simulink model "mcb_microchip_pmsm_parameter_est_SAME70"  (R2023b)
settings: Solver=FixedStepDiscrete  StartTime=0.0  StopTime=15  RelTol=1e-3  EnableMultiTasking=on
InitFcn:
  | mcb_microchip_pmsm_parameter_est_SAME70_data;
values from neighbouring files (symbols this model uses):
  Ts = T_pwm    (= 5e-05)    [mcb_microchip_pmsm_parameter_est_SAME70_data.m]
  Ts_motor = T_pwm/2    (= 2.5e-05)    [mcb_microchip_pmsm_parameter_est_SAME70_data.m]
undefined symbols (not defined in the file or in its folder): A24, AD10, AD7, ADC0, inverter, LQFP144, MaxPer, ms, ns, PA0, PA1, PA10, PA11, PA12, PA13, PA16, PA18, PA9, PB0, PD18, PD19, PD24, PD25, PD26, PI_params, Pin, pmsm, Resol, SAME70Q21B, target, Unsigned
libraries: simulink x18, MCHP_Blockset x13, mcbpmsmparamestlib x5, svdutilitieslib x4, mcbpositiondecoderlib x3, mcbplantlib x1, autolibpmsmexterior x1, mcbcontrolslib x1
(part 2 of 4)

== system mcb_microchip_pmsm_parameter_est_SAME70/Microcontroller/Configurations ==
  note: PIM: https://www.microchip.com/Developmenttools/ProductDetails/MA320203
  note: MCLV-2				SAME70-PIM
      | --------------------------------------------------
      | DBG_LED1			PC23
      | DBG_LED2			PA24
      |
      | Rx					PA09_URXD0
      | Tx					PA10_UTXD0
      |
      | HALLA				PA00 - PD13
      | HALLB				PA01 - PD10
      | HALLC				PA16 - PD11
      |
      | PWM1				PD24 (L) - PA11 (H)
      | PWM2				PD25 (L) - PA12 (H)
      | PWM3				PD26 (L) - PA13 (H)
      |
      | FAULT				PD09_FAULT_PWM
      |
      | POT				PB00 (not ok on early PIMs)
      | PUSH S2			PC03
      | PUSH S3			PC01
      |
      | PIM_V_M1			PD30
      | PIM_V_M2			PA17
      | PIM_V_M3			PA21 - PA19
  Compiler Options : MCHP_Blockset/System Configuration/Compiler Options  Priority=1  LATEST_CMPLR=on  COMP_LIST=Dynamic Options  COMP_LIST_TXT=xc32 - v4.30  DFP_LIST=Dynamic Options  DFP_LIST_TXT=from compiler  CMSIS_DSP=Dynamic Options  CMSIS_DSP_TXT=Not used  USE_64BIT_DOUBLE=off  MCHP_MULTITHREAD_COMPILATION=on  UseCustom_LinkerScript=off  MCHP_MASTERLINK=mcb_microchip_pmsm_parameter_est_SAME70_23b_lib/Microcontroller/Configurations/Microchip Master  OPTIMIZATION_LEVEL=2  MPLAB_LINKLIB=default  MPLAB_LINKLIB1=default  CodeReplacement=Dynamic Options  CodeReplacement_TXT=None  OPTIMIZATION_FLTO=off  OPTIMIZATION_REORDER=off  UNROLL_LOOPS=off  PROCEDURAL_ABSTRACTION=off  MCODE=is less than 32768 (faster)  MCONST=in data memory  MDATA=Use only memory below address 8192 (faster)  MSCALAR=Use only memory below address 8192 (faster)  MLARGEARRAY=off  MAGGREGATE=off  HEAP_SIZE=0  OMF=elf  DEBUG_INFO=on  ProduceHexOutput=off  AssemblyListing=off  SaveTemps=off  NO_EDS_WARN=on  PRINT_STATISTICS=off
      settings: SourceProductName=MPLAB Device Blocks for Simulink
  Microchip Master : MCHP_Blockset/System Configuration/Microchip Master  Priority=1  PICREF=SAME70Q21B - LQFP144  TIMESTEP_REF="ADC0  ( 0.001s )"  BUSYFLAG=Dynamic Options  BUSYFLAG_TXT=A24 / Pin[56]  VDD_range=Dynamic Options  PWRTEN=Not used  BOREN=Disable  BODENV=2.7V  BORV=Not used  FPWRT=64ms  DSBOREN=Enable ZPBOR during Deep Sleep Mode  DSLPBOR=Not used  MCLRE=Enabled  SMCLR=MCLR pin generates a normal system Reset  PMDL1WAY=Allow only one reconfiguration  RSTPRI=Device will obtain reset instruction from Primary flash  TEMP=Not used  SOSCSRC=Not used  SOSCSEL=Not used  IOL1WAY=Allow only one reconfiguration  ALTVREF=Not used  DISUVREG=Not used  DSSWEN=Not used  LPCFG=Not used  RTCBAT=Not used  VBTBOR=Not used  WUTSEL=Not used  POWERSAVE=off  FNOSC=Fast RC Osc w/Div-by-N (FRCDIV)  FPR=ECIO w/ PLL 16x  FOSFPR=HS3 w/PLL 16x  FOS=Internal Fast RC  FRANGE=High Range  OSCILLATOR_SELECT=Crystal / Ceramic resonator  OSCILLATOR_SELECT_spd=Crystal / Ceramic resonator  QUARTZ=12e6  QUARTZ_spd=12e6  POSCGAIN=2x gain setting  POSCBOOST=Boost the kick start of the oscillator  SOSCGAIN=2x gain setting  SOSCBOOST=Boost the kick start of the oscillator  ACTIV_PLL=on  ACTIV_PLL_spd=on  MIPS_DESIRED=300e6  MIPS_DESIRED_spd=300e6  CPUDIV=Divide by 1  FPLLMUL=Not used  FPLLIDIV=8x Divider  POSCFREQ=Not used  POSCMD=Primary Oscillator Disabled  POSCMOD=Primary osc disabled  MIPS=300 * 1e6  ACLKCON=Optimized for PWM resolution & ADC conversion speed  ACLKCON_spd=Optimized for PWM resolution & ADC conversion speed  FPLLODIV=32x Divider  PLLKEN=Clock switch to PLL source will wait until the PLL lock signal is valid  FCKSM=Clock Switch Disabled; FSCM Disabled  FCKSMEN=Sw Disabled; Mon Disabled  IESO=Enabled  DSWDTPS=1:2^36  FWDTEN=Disable  FWDTWINSZ=Window size is 25%  FWPSA=1:512  FWPSA0=1:128  FWPSB=1:16  WDT=Disable  WDTPOST=1:32768  WDTPRE=1:128  WDTPS=1:1048576  WINDIS=Watchdog Timer is in non-Window mode  WWDTEN=Non-Window mode  DSWDTEN=Enable DSWDT during Deep Sleep Mode  DSWDTOSC=Select LPRC as DSWDT Reference clock  FWDT_RCLKSEL=WDT Run Mode uses BFRC:256  FWDT_RWDTPS=1:2147483648  FWDT_SWDTMPS=1:2147483648  FWDT_WDTEN=WDT is controlled by software; use WDTCON.ON bit  FWDT_WDTRSTEN=WDT event generates a reset  FWDT_WDTWIN=WDT Window is 25% of WDT period  FWDT_WINEN=Watchdog Timer operates in Window mode  FPBDIV=Not used  FSOSCEN=Disable Secondary Oscillator  LPRCSEL=Not used  OSCIOFCN=Not used  OSCIOFNC=OSC2 is clock output  LVRCFG=Not used  PLL_96MHZ=Not used  PLL96MHZ=Not used  PLLDIV=Not used  WDTCLK=Not used  WDTCMX=Not used  WDTWIN=WDT Window is 25% of WDT period  XTCFG=24-32 MHz crystals  XTBST=Boost the kick-start  APL=Aux Flash Code protect is disabled  APLK=Aux Flash Write Protection or Code Protection is Enabled  AWRP=Auxiliary program memory is not write-protected  BSS=No Boot program Flash segment  BWP=Not used  BWRP=Boot Segment may be written  CP=Protection Disabled  EBS=No Boot EEPROM  ESS=No Segment Data EEPROM  GCP=Disable  GSS=High Security Code Protection Enabled  GSS0=Not used  GSSK=General Segment Write Protection or Code Protection is Enabled  GWRP=Disable  PWP=Not used  RBS=No Boot RAM  RSS=No Secure RAM  SSS=No Secure Segment  SWRP=Secure segment may be written  WPCFG=Not used  WPDIS=Not used  WPEND=Not used  WPFP=Not used  ICESEL=Communicate on PGEC1/PGED1  ICS=Use PGC/EMUC and PGD/EMUD  JTAGEN=Disable  FICD_JTAGEN=Disable  COE=Not used  RES=Not used  DEBUG=Debugger is disabled  BACKBUG=Not used  BKBUG=Not used  ALTI2C=I2C mapped to SDA1/SCL1 pins  ALTI2C1=I2C1 mapped to SDA1/SCL1 pins  ALTI2C2=I2C2 mapped to SDA2/SCL2 pins  ALTI2C3=I2C3 mapped to SDA3/SCL3 pins  FDEVOPT1_ALTI2C1=Primary I2C1 pins are used  FDEVOPT1_ALTI2C2=Primary I2C2 pins are used  FDEVOPT1_SPI2MAPDIS=SPI2 pins are selected by peripheral pin selection feature  ALTQIO=QEA1; QEB1; INDX1 are selected as inputs to QEI1  ALTSS1=SS1A is selected as the I/O pin for SPI1  CMPPOL0=Hysteresis is applied to falling edge  CMPPOL1=Hysteresis is applied to falling edge  FCANIO=Not used  FETHIO=Default Ethernet I/O  FMIIEN=MII Enabled  FSRSSEL=Not used  FUSBIDIO=Controlled by the USB Module  FVBUSONIO=Not used  HPOL=Active High  HYST0=45 mV Hysteresis  HYST1=45 mV Hysteresis  I2C1SEL=Not used  LPOL=Active High  PWMPIN=Control with PORT/TRIS regs  RTCOSC=Not used  UPLLEN=USB PLL Disabled  UPLLIDIV=Not used  ATMOD8=Not used  ALTPMP=Not used  I2C2SEL=Not used  ALTADREF=Not used  ALTCVREF=Not used  PWMLOCK=PWM registers may be written without key sequence  INT_PRIORITY_DMA=7  MCHP_TIMER_RESULT=[1 98.999999999999971578 ]  MCHP_PORT={Busy Flag}{Busy}0:1:A24;  MCHP_PLLRegisters=[-1 -1 -1 -1 -1]  MCHPVAR=MCHP.id.name='SAME70Q21B';MCHP.id.N=reshape([70 21 -1],1,3);MCHP.id.L=reshape({ 'SAME','Q','B'},1,3);MCHP.id.maskset='';MCHP.id.dos='';MCHP.id.ds='';MCHP.id.archTxt='';MCHP.id.clonedfrom='';MCHP.id.Arch=5;MCHP.id.pinout=reshape({ 'LFBGA144','UFBGA144','LQFP144'},1,3);MCHP.Rx=reshape([102 21 11 1 4 99 20 38 132 6 93 26 39 131 7 91 31 40 128 10 77 105 41 126 27 73 109 58 125 28 114 79 54 121 -1 35 89 48 119 -1 36 141 82 113 -1 75 142 86 110 -1 66 -1 90 101 -1 64 -1 94 98 -1 68 87 17 92 -1 42 144 19 88 -1 51 -1 97 84 -1 49 -1 18 106 -1 45 -1 100 78 -1 25 -1 103 74 -1 24 -1 111 69 -1 23 -1 117 67 -1 22 -1 120 65 -1 32 -1 122 63 -1 37 -1 124 60 -1 46 -1 127 57 -1 56 -1 130 55 -1 59 -1 133 52 -1 62 -1 13 53 -1 70 -1 12 47 -1 112 -1 76 71 -1 129 -1 16 108 -1 116 -1 15 34 -1 118 -1 14 2 -1],5,32);MCHP.memory.PERIPHERALS.size=MCHP_Fun.Hex2num('41C0000000000000');MCHP.memory.SYSTEM.size=MCHP_Fun.Hex2num('41B0000000000000');MCHP.memory.QSPIMEM.size=MCHP_Fun.Hex2num('41C0000000000000');MCHP.memory.AXIMX.size=1048576;MCHP.memory.ITCM.size=2097152;MCHP.memory.IFLASH.size=2097152;MCHP.memory.IROM.size=16384;MCHP.memory.DTCM.size=131072;MCHP.memory.IRAM.size=393216;MCHP.memory.EBI_CS0.size=16777216;MCHP.memory.EBI_CS1.size=16777216;MCHP.memory.EBI_CS2.size=16777216;MCHP.memory.EBI_CS3.size=16777216;MCHP.module.SUPC.PID=0;MCHP.module.SUPC.vector='SUPC';MCHP.module.SUPC.pin.WKUP0.txt={ 'PA0'};MCHP.module.SUPC.pin.WKUP0.Rx_idx=0;MCHP.module.SUPC.pin.WKUP0.ABCD=-2;MCHP.module.SUPC.pin.WKUP1.txt={ 'PA1'};MCHP.module.SUPC.pin.WKUP1.Rx_idx=1;MCHP.module.SUPC.pin.WKUP1.ABCD=-2;MCHP.module.SUPC.pin.WKUP2.txt={ 'PA2'};MCHP.module.SUPC.pin.WKUP2.Rx_idx=2;MCHP.module.SUPC.pin.WKUP2.ABCD=-2;MCHP.module.SUPC.pin.WKUP3.txt={ 'PA4'};MCHP.module.SUPC.pin.WKUP3.Rx_idx=4;MCHP.module.SUPC.pin.WKUP3.ABCD=-2;MCHP.module.SUPC.pin.WKUP4.txt={ 'PA5'};MCHP.module.SUPC.pin.WKUP4.Rx_idx=5;MCHP.module.SUPC.pin.WKUP4.ABCD=-2;MCHP.module.SUPC.pin.WKUP6.txt={ 'PA9'};MCHP.module.SUPC.pin.WKUP6.Rx_idx=9;MCHP.module.SUPC.pin.WKUP6.ABCD=-2;MCHP.module.SUPC.pin.WKUP7.txt={ 'PA11'};MCHP.module.SUPC.pin.WKUP7.Rx_idx=11;MCHP.module.SUPC.pin.WKUP7.ABCD=-2;MCHP.module.SUPC.pin.WKUP8.txt={ 'PA14'};MCHP.module.SUPC.pin.WKUP8.Rx_idx=14;MCHP.module.SUPC.pin.WKUP8.ABCD=-2;MCHP.module.SUPC.pin.WKUP9.txt={ 'PA19'};MCHP.module.SUPC.pin.WKUP9.Rx_idx=19;MCHP.module.SUPC.pin.WKUP9.ABCD=-2;MCHP.module.SUPC.pin.WKUP10.txt={ 'PA20'};MCHP.module.SUPC.pin.WKUP10.Rx_idx=20;MCHP.module.SUPC.pin.WKUP10.ABCD=-2;MCHP.module.SUPC.pin.WKUP11.txt={ 'PA30'};MCHP.module.SUPC.pin.WKUP11.Rx_idx=30;MCHP.module.SUPC.pin.WKUP11.ABCD=-2;MCHP.module.SUPC.pin.WKUP12.txt={ 'PB3'};MCHP.module.SUPC.pin.WKUP12.Rx_idx=35;MCHP.module.SUPC.pin.WKUP12.ABCD=-2;MCHP.module.SUPC.pin.WKUP13.txt={ 'PB5'};MCHP.module.SUPC.pin.WKUP13.Rx_idx=37;MCHP.module.SUPC.pin.WKUP13.ABCD=-2;MCHP.module.SUPC.pin.WKUP5.txt={ 'PD28'};MCHP.module.SUPC.pin.WKUP5.Rx_idx=124;MCHP.module.SUPC.pin.WKUP5.ABCD=-2;MCHP.module.RSTC.PID=1;MCHP.module.RSTC.vector='RSTC';MCHP.module.RTC.PID=2;MCHP.module.RTC.vector='RTC';MCHP.module.RTC.pin.RTCOUT0.txt={ 'PB0'};MCHP.module.RTC.pin.RTCOUT0.Rx_idx=32;MCHP.module.RTC.pin.RTCOUT0.ABCD=-2;MCHP.module.RTC.pin.RTCOUT1.txt={ 'PB1'};MCHP.module.RTC.pin.RTCOUT1.Rx_idx=33;MCHP.module.RTC.pin.RTCOUT1.ABCD=-2;MCHP.module.RTT.PID=3;MCHP.module.RTT.vector='RTT';MCHP.module.WDT.PID=4;MCHP.module.WDT.vector='WDT';MCHP.module.PMC.PID=5;MCHP.module.PMC.vector='PMC';MCHP.module.PMC.pin.PCK0.txt=reshape({ 'PA6','PB12','PB13'},1,3);MCHP.module.PMC.pin.PCK0.Rx_idx=reshape([6 44 45],1,3);MCHP.module.PMC.pin.PCK0.ABCD=reshape([1 3 1],1,3);MCHP.module.PMC.pin.PCK1.txt=reshape({ 'PA17','PA21'},1,2);MCHP.module.PMC.pin.PCK1.Rx_idx=reshape([17 21],1,2);MCHP.module.PMC.pin.PCK1.ABCD=reshape([1 1],1,2);MCHP.module.PMC.pin.PCK2.txt=reshape({ 'PA3','PA18','PA31','PB3','PD31'},1,5);MCHP.module.PMC.pin.PCK2.Rx_idx=reshape([3 18 31 35 127],1,5);MCHP.module.PMC.pin.PCK2.ABCD=reshape([2 1 1 1 2],1,5);MCHP.module.PMC.pin.XIN.txt={ 'PB9'};MCHP.module.PMC.pin.XIN.Rx_idx=41;MCHP.module.PMC.pin.XIN.ABCD=-2;MCHP.module.PMC.pin.XOUT.txt={ 'PB8'};MCHP.module.PMC.pin.XOUT.Rx_idx=40;MCHP.module.PMC.pin.XOUT.ABCD=-2;MCHP.module.PMC.pin.XIN32.txt={ 'PA7'};MCHP.module.PMC.pin.XIN32.Rx_idx=7;MCHP.module.PMC.pin.XIN32.ABCD=-2;MCHP.module.PMC.pin.XOUT32.txt={ 'PA8'};MCHP.module.PMC.pin.XOUT32.Rx_idx=8;MCHP.module.PMC.pin.XOUT32.ABCD=-2;MCHP.module.EFC.PID=6;MCHP.module.EFC.vector='EFC';MCHP.module.EFC.pin.ERASE.txt={ 'PB12'};MCHP.module.EFC.pin.ERASE.Rx_idx=44;MCHP.module.EFC.pin.ERASE.ABCD=-2;MCHP.module.UART0.PID=7;MCHP.module.UART0.vector='UART0';MCHP.module.UART0.pin.URXD0.txt={ 'PA9'};MCHP.module.UART0.pin.URXD0.Rx_idx=9;MCHP.module.UART0.pin.URXD0.ABCD=0;MCHP.module.UART0.pin.UTXD0.txt={ 'PA10'};MCHP.module.UART0.pin.UTXD0.Rx_idx=10;MCHP.module.UART0.pin.UTXD0.ABCD=0;MCHP.module.UART1.PID=8;MCHP.module.UART1.vector='UART1';MCHP.module.UART1.pin.URXD1.txt={ 'PA5'};MCHP.module.UART1.pin.URXD1.Rx_idx=5;MCHP.module.UART1.pin.URXD1.ABCD=2;MCHP.module.UART1.pin.UTXD1.txt=reshape({ 'PA4','PA6','PD26'},1,3);MCHP.module.UART1.pin.UTXD1.Rx_idx=reshape([4 6 122],1,3);MCHP.module.UART1.pin.UTXD1.ABCD=reshape([2 2 3],1,3);MCHP.module.PIOA.PID=10;MCHP.module.PIOA.vector='PIOA';MCHP.module.PIOA.pin.PIODC0.txt={ 'PA3'};MCHP.module.PIOA.pin.PIODC0.Rx_idx=3;MCHP.module.PIOA.pin.PIODC0.ABCD=-2;MCHP.module.PIOA.pin.PIODC1.txt={ 'PA4'};MCHP.module.PIOA.pin.PIODC1.Rx_idx=4;MCHP.module.PIOA.pin.PIODC1.ABCD=-2;MCHP.module.PIOA.pin.PIODC2.txt={ 'PA5'};MCHP.module.PIOA.pin.PIODC2.Rx_idx=5;MCHP.module.PIOA.pin.PIODC2.ABCD=-2;MCHP.module.PIOA.pin.PIODC3.txt={ 'PA9'};MCHP.module.PIOA.pin.PIODC3.Rx_idx=9;MCHP.module.PIOA.pin.PIODC3.ABCD=-2;MCHP.module.PIOA.pin.PIODC4.txt={ 'PA10'};MCHP.module.PIOA.pin.PIODC4.Rx_idx=10;MCHP.module.PIOA.pin.PIODC4.ABCD=-2;MCHP.module.PIOA.pin.PIODC5.txt={ 'PA11'};MCHP.module.PIOA.pin.PIODC5.Rx_idx=11;MCHP.module.PIOA.pin.PIODC5.ABCD=-2;MCHP.module.PIOA.pin.PIODC6.txt={ 'PA12'};MCHP.module.PIOA.pin.PIODC6.Rx_idx=12;MCHP.module.PIOA.pin.PIODC6.ABCD=-2;MCHP.module.PIOA.pin.PIODC7.txt={ 'PA13'};MCHP.module.PIOA.pin.PIODC7.Rx_idx=13;MCHP.module.PIOA.pin.PIODC7.ABCD=-2;MCHP.module.PIOA.pin.PIODCEN1.txt={ 'PA14'};MCHP.module.PIOA.pin.PIODCEN1.Rx_idx=14;MCHP.module.PIOA.pin.PIODCEN1.ABCD=-2;MCHP.module.PIOA.pin.PIODCEN2.txt={ 'PA21'};MCHP.module.PIOA.pin.PIODCEN2.Rx_idx=21;MCHP.module.PIOA.pin.PIODCEN2.ABCD=-2;MCHP.module.PIOA.pin.PIODCCLK.txt={ 'PA22'};MCHP.module.PIOA.pin.PIODCCLK.Rx_idx=22;MCHP.module.PIOA.pin.PIODCCLK.ABCD=-2;MCHP.module.PIOB.PID=11;MCHP.module.PIOB.vector='PIOB';MCHP.module.PIOC.PID=12;MCHP.module.PIOC.vector='PIOC';MCHP.module.USART0.PID=13;MCHP.module.USART0.vector='USART0';MCHP.module.USART0.pin.CTS0.txt={ 'PB2'};MCHP.module.USART0.pin.CTS0.Rx_idx=34;MCHP.module.USART0.pin.CTS0.ABCD=2;MCHP.module.USART0.pin.DCD0.txt={ 'PD0'};MCHP.module.USART0.pin.DCD0.Rx_idx=96;MCHP.module.USART0.pin.DCD0.ABCD=3;MCHP.module.USART0.pin.DSR0.txt={ 'PD2'};MCHP.module.USART0.pin.DSR0.Rx_idx=98;MCHP.module.USART0.pin.DSR0.ABCD=3;MCHP.module.USART0.pin.DTR0.txt={ 'PD1'};MCHP.module.USART0.pin.DTR0.Rx_idx=97;MCHP.module.USART0.pin.DTR0.ABCD=3;MCHP.module.USART0.pin.RI0.txt={ 'PD3'};MCHP.module.USART0.pin.RI0.Rx_idx=99;MCHP.module.USART0.pin.RI0.ABCD=3;MCHP.module.USART0.pin.RTS0.txt={ 'PB3'};MCHP.module.USART0.pin.RTS0.Rx_idx=35;MCHP.module.USART0.pin.RTS0.ABCD=2;MCHP.module.USART0.pin.RXD0.txt={ 'PB0'};MCHP.module.USART0.pin.RXD0.Rx_idx=32;MCHP.module.USART0.pin.RXD0.ABCD=2;MCHP.module.USART0.pin.SCK0.txt={ 'PB13'};MCHP.module.USART0.pin.SCK0.Rx_idx=45;MCHP.module.USART0.pin.SCK0.ABCD=2;MCHP.module.USART0.pin.TXD0.txt={ 'PB1'};MCHP.module.USART0.pin.TXD0.Rx_idx=33;MCHP.module.USART0.pin.TXD0.ABCD=2;MCHP.module.USART1.PID=14;MCHP.module.USART1.vector='USART1';MCHP.module.USART1.pin.CTS1.txt={ 'PA25'};MCHP.module.USART1.pin.CTS1.Rx_idx=25;MCHP.module.USART1.pin.CTS1.ABCD=0;MCHP.module.USART1.pin.DCD1.txt={ 'PA26'};MCHP.module.USART1.pin.DCD1.Rx_idx=26;MCHP.module.USART1.pin.DCD1.ABCD=0;MCHP.module.USART1.pin.DSR1.txt={ 'PA28'};MCHP.module.USART1.pin.DSR1.Rx_idx=28;MCHP.module.USART1.pin.DSR1.ABCD=0;MCHP.module.USART1.pin.DTR1.txt={ 'PA27'};MCHP.module.USART1.pin.DTR1.Rx_idx=27;MCHP.module.USART1.pin.DTR1.ABCD=0;MCHP.module.USART1.pin.LONCOL1.txt={ 'PA3'};MCHP.module.USART1.pin.LONCOL1.Rx_idx=3;MCHP.module.USART1.pin.LONCOL1.ABCD=1;MCHP.module.USART1.pin.RI1.txt={ 'PA29'};MCHP.module.USART1.pin.RI1.Rx_idx=29;MCHP.module.USART1.pin.RI1.ABCD=0;MCHP.module.USART1.pin.RTS1.txt={ 'PA24'};MCHP.module.USART1.pin.RTS1.Rx_idx=24;MCHP.module.USART1.pin.RTS1.ABCD=0;MCHP.module.USART1.pin.RXD1.txt={ 'PA21'};MCHP.module.USART1.pin.RXD1.Rx_idx=21;MCHP.module.USART1.pin.RXD1.ABCD=0;MCHP.module.USART1.pin.SCK1.txt={ 'PA23'};MCHP.module.USART1.pin.SCK1.Rx_idx=23;MCHP.module.USART1.pin.SCK1.ABCD=0;MCHP.module.USART1.pin.TXD1.txt={ 'PB4'};MCHP.module.USART1.pin.TXD1.Rx_idx=36;MCHP.module.USART1.pin.TXD1.ABCD=3;MCHP.module.USART2.PID=15;MCHP.module.USART2.vector='USART2';MCHP.module.USART2.pin.CTS2.txt={ 'PD19'};MCHP.module.USART2.pin.CTS2.Rx_idx=115;MCHP.module.USART2.pin.CTS2.ABCD=1;MCHP.module.USART2.pin.DCD2.txt={ 'PD4'};MCHP.module.USART2.pin.DCD2.Rx_idx=100;MCHP.module.USART2.pin.DCD2.ABCD=3;MCHP.module.USART2.pin.DSR2.txt={ 'PD6'};MCHP.module.USART2.pin.DSR2.Rx_idx=102;MCHP.module.USART2.pin.DSR2.ABCD=3;MCHP.module.USART2.pin.DTR2.txt={ 'PD5'};MCHP.module.USART2.pin.DTR2.Rx_idx=101;MCHP.module.USART2.pin.DTR2.ABCD=3;MCHP.module.USART2.pin.RI2.txt={ 'PD7'};MCHP.module.USART2.pin.RI2.Rx_idx=103;MCHP.module.USART2.pin.RI2.ABCD=3;MCHP.module.USART2.pin.RTS2.txt={ 'PD18'};MCHP.module.USART2.pin.RTS2.Rx_idx=114;MCHP.module.USART2.pin.RTS2.ABCD=1;MCHP.module.USART2.pin.RXD2.txt={ 'PD15'};MCHP.module.USART2.pin.RXD2.Rx_idx=111;MCHP.module.USART2.pin.RXD2.ABCD=1;MCHP.module.USART2.pin.SCK2.txt={ 'PD17'};MCHP.module.USART2.pin.SCK2.Rx_idx=113;MCHP.module.USART2.pin.SCK2.ABCD=1;MCHP.module.USART2.pin.TXD2.txt={ 'PD16'};MCHP.module.USART2.pin.TXD2.Rx_idx=112;MCHP.module.USART2.pin.TXD2.ABCD=1;MCHP.module.PIOD.PID=16;MCHP.module.PIOD.vector='PIOD';MCHP.module.PIOE.PID=17;MCHP.module.PIOE.vector='PIOE';MCHP.module.HSMCI.PID=18;MCHP.module.HSMCI.vector='HSMCI';MCHP.module.HSMCI.pin.MCCDA.txt={ 'PA28'};MCHP.module.HSMCI.pin.MCCDA.Rx_idx=28;MCHP.module.HSMCI.pin.MCCDA.ABCD=2;MCHP.module.HSMCI.pin.MCCK.txt={ 'PA25'};MCHP.module.HSMCI.pin.MCCK.Rx_idx=25;MCHP.module.HSMCI.pin.MCCK.ABCD=3;MCHP.module.HSMCI.pin.MCDA0.txt={ 'PA30'};MCHP.module.HSMCI.pin.MCDA0.Rx_idx=30;MCHP.module.HSMCI.pin.MCDA0.ABCD=2;MCHP.module.HSMCI.pin.MCDA1.txt={ 'PA31'};MCHP.module.HSMCI.pin.MCDA1.Rx_idx=31;MCHP.module.HSMCI.pin.MCDA1.ABCD=2;MCHP.module.HSMCI.pin.MCDA2.txt={ 'PA26'};MCHP.module.HSMCI.pin.MCDA2.Rx_idx=26;MCHP.module.HSMCI.pin.MCDA2.ABCD=2;MCHP.module.HSMCI.pin.MCDA3.txt={ 'PA27'};MCHP.module.HSMCI.pin.MCDA3.Rx_idx=27;MCHP.module.HSMCI.pin.MCDA3.ABCD=2;MCHP.module.TWIHS0.PID=19;MCHP.module.TWIHS0.vector='TWIHS0';MCHP.module.TWIHS0.pin.TWCK0.txt={ 'PA4'};MCHP.module.TWIHS0.pin.TWCK0.Rx_idx=4;MCHP.module.TWIHS0.pin.TWCK0.ABCD=0;MCHP.module.TWIHS0.pin.TWD0.txt={ 'PA3'};MCHP.module.TWIHS0.pin.TWD0.Rx_idx=3;MCHP.module.TWIHS0.pin.TWD0.ABCD=0;MCHP.module.TWIHS1.PID=20;MCHP.module.TWIHS1.vector='TWIHS1';MCHP.module.TWIHS1.pin.TWCK1.txt={ 'PB5'};MCHP.module.TWIHS1.pin.TWCK1.Rx_idx=37;MCHP.module.TWIHS1.pin.TWCK1.ABCD=0;MCHP.module.TWIHS1.pin.TWD1.txt={ 'PB4'};MCHP.module.TWIHS1.pin.TWD1.Rx_idx=36;MCHP.module.TWIHS1.pin.TWD1.ABCD=0;MCHP.module.SPI0.PID=21;MCHP.module.SPI0.vector='SPI0';MCHP.module.SPI0.pin.MISO.txt={ 'PD20'};MCHP.module.SPI0.pin.MISO.Rx_idx=116;MCHP.module.SPI0.pin.MISO.ABCD=1;MCHP.module.SPI0.pin.MOSI.txt={ 'PD21'};MCHP.module.SPI0.pin.MOSI.Rx_idx=117;MCHP.module.SPI0.pin.MOSI.ABCD=1;MCHP.module.SPI0.pin.NPCS0.txt={ 'PB2'};MCHP.module.SPI0.pin.NPCS0.Rx_idx=34;MCHP.module.SPI0.pin.NPCS0.ABCD=3;MCHP.module.SPI0.pin.NPCS1.txt=reshape({ 'PA31','PD25'},1,2);MCHP.module.SPI0.pin.NPCS1.Rx_idx=reshape([31 121],1,2);MCHP.module.SPI0.pin.NPCS1.ABCD=reshape([0 1],1,2);MCHP.module.SPI0.pin.NPCS2.txt={ 'PD12'};MCHP.module.SPI0.pin.NPCS2.Rx_idx=108;MCHP.module.SPI0.pin.NPCS2.ABCD=2;MCHP.module.SPI0.pin.NPCS3.txt={ 'PD27'};MCHP.module.SPI0.pin.NPCS3.Rx_idx=123;MCHP.module.SPI0.pin.NPCS3.ABCD=1;MCHP.module.SPI0.pin.SPCK.txt={ 'PD22'};MCHP.module.SPI0.pin.SPCK.Rx_idx=118;MCHP.module.SPI0.pin.SPCK.ABCD=1;MCHP.module.SSC.PID=22;MCHP.module.SSC.vector='SSC';MCHP.module.SSC.pin.RD.txt={ 'PA10'};MCHP.module.SSC.pin.RD.Rx_idx=10;MCHP.module.SSC.pin.RD.ABCD=2;MCHP.module.SSC.pin.RF.txt={ 'PD24'};MCHP.module.SSC.pin.RF.Rx_idx=120;MCHP.module.SSC.pin.RF.ABCD=1;MCHP.module.SSC.pin.RK.txt={ 'PA22'};MCHP.module.SSC.pin.RK.Rx_idx=22;MCHP.module.SSC.pin.RK.ABCD=0;MCHP.module.SSC.pin.TD.txt=reshape({ 'PB5','PD10','PD26'},1,3);MCHP.module.SSC.pin.TD.Rx_idx=reshape([37 106 122],1,3);MCHP.module.SSC.pin.TD.ABCD=reshape([3 2 1],1,3);MCHP.module.SSC.pin.TF.txt={ 'PB0'};MCHP.module.SSC.pin.TF.Rx_idx=32;MCHP.module.SSC.pin.TF.ABCD=3;MCHP.module.SSC.pin.TK.txt={ 'PB1'};MCHP.module.SSC.pin.TK.Rx_idx=33;MCHP.module.SSC.pin.TK.ABCD=3;MCHP.module.TC0(1).PID=23;MCHP.module.TC0(1).vector='TC0';MCHP.module.TC0(1).pin.TCLK0.txt={ 'PA4'};MCHP.module.TC0(1).pin.TCLK0.Rx_idx=4;MCHP.module.TC0(1).pin.TCLK0.ABCD=1;MCHP.module.TC0(1).pin.TCLK1.txt={ 'PA28'};MCHP.module.TC0(1).pin.TCLK1.Rx_idx=28;MCHP.module.TC0(1).pin.TCLK1.ABCD=1;MCHP.module.TC0(1).pin.TCLK2.txt={ 'PA29'};MCHP.module.TC0(1).pin.TCLK2.Rx_idx=29;MCHP.module.TC0(1).pin.TCLK2.ABCD=1;MCHP.module.TC0(1).pin.TIOA0.txt={ 'PA0'};MCHP.module.TC0(1).pin.TIOA0.Rx_idx=0;MCHP.module.TC0(1).pin.TIOA0.ABCD=1;MCHP.module.TC0(1).pin.TIOA1.txt={ 'PA15'};MCHP.module.TC0(1).pin.TIOA1.Rx_idx=15;MCHP.module.TC0(1).pin.TIOA1.ABCD=1;MCHP.module.TC0(1).pin.TIOA2.txt={ 'PA26'};MCHP.module.TC0(1).pin.TIOA2.Rx_idx=26;MCHP.module.TC0(1).pin.TIOA2.ABCD=1;MCHP.module.TC0(1).pin.TIOB0.txt={ 'PA1'};MCHP.module.TC0(1).pin.TIOB0.Rx_idx=1;MCHP.module.TC0(1).pin.TIOB0.ABCD=1;MCHP.module.TC0(1).pin.TIOB1.txt={ 'PA16'};MCHP.module.TC0(1).pin.TIOB1.Rx_idx=16;MCHP.module.TC0(1).pin.TIOB1.ABCD=1;MCHP.module.TC0(1).pin.TIOB2.txt={ 'PA27'};MCHP.module.TC0(1).pin.TIOB2.Rx_idx=27;MCHP.module.TC0(1).pin.TIOB2.ABCD=1;MCHP.module.TC0(2).PID=24;MCHP.module.TC0(2).vector='TC1';MCHP.module.TC0(2).pin=reshape(MCHP_Fun.Hex2num('[]'),0,0);MCHP.module.TC0(3).PID=25;MCHP.module.TC0(3).vector='TC2';MCHP.module.TC0(3).pin=reshape(MCHP_Fun.Hex2num('[]'),0,0);MCHP.module.TC1(1).PID=26;MCHP.module.TC1(1).vector='TC3';MCHP.module.TC1(1).pin.TCLK3.txt={ 'PC25'};MCHP.module.TC1(1).pin.TCLK3.Rx_idx=89;MCHP.module.TC1(1).pin.TCLK3.ABCD=1;MCHP.module.TC1(1).pin.TCLK4.txt={ 'PC28'};MCHP.module.TC1(1).pin.TCLK4.Rx_idx=92;MCHP.module.TC1(1).pin.TCLK4.ABCD=1;MCHP.module.TC1(1).pin.TCLK5.txt={ 'PC31'};MCHP.module.TC1(1).pin.TCLK5.Rx_idx=95;MCHP.module.TC1(1).pin.TCLK5.ABCD=1;MCHP.module.TC1(1).pin.TIOA3.txt={ 'PC23'};MCHP.module.TC1(1).pin.TIOA3.Rx_idx=87;MCHP.module.TC1(1).pin.TIOA3.ABCD=1;MCHP.module.TC1(1).pin.TIOA4.txt={ 'PC26'};MCHP.module.TC1(1).pin.TIOA4.Rx_idx=90;MCHP.module.TC1(1).pin.TIOA4.ABCD=1;MCHP.module.TC1(1).pin.TIOA5.txt={ 'PC29'};MCHP.module.TC1(1).pin.TIOA5.Rx_idx=93;MCHP.module.TC1(1).pin.TIOA5.ABCD=1;MCHP.module.TC1(1).pin.TIOB3.txt={ 'PC24'};MCHP.module.TC1(1).pin.TIOB3.Rx_idx=88;MCHP.module.TC1(1).pin.TIOB3.ABCD=1;MCHP.module.TC1(1).pin.TIOB4.txt={ 'PC27'};MCHP.module.TC1(1).pin.TIOB4.Rx_idx=91;MCHP.module.TC1(1).pin.TIOB4.ABCD=1;MCHP.module.TC1(1).pin.TIOB5.txt={ 'PC30'};MCHP.module.TC1(1).pin.TIOB5.Rx_idx=94;MCHP.module.TC1(1).pin.TIOB5.ABCD=1;MCHP.module.TC1(2).PID=27;MCHP.module.TC1(2).vector='TC4';MCHP.module.TC1(2).pin=reshape(MCHP_Fun.Hex2num('[]'),0,0);MCHP.module.TC1(3).PID=28;MCHP.module.TC1(3).vector='TC5';MCHP.module.TC1(3).pin=reshape(MCHP_Fun.Hex2num('[]'),0,0);MCHP.module.AFEC0.PID=29;MCHP.module.AFEC0.vector='AFEC0';MCHP.module.AFEC0.pin.ADTRG.txt={ 'PA8'};MCHP.module.AFEC0.pin.ADTRG.Rx_idx=8;MCHP.module.AFEC0.pin.ADTRG.ABCD=1;MCHP.module.AFEC0.pin.AD0.txt={ 'PD30'};MCHP.module.AFEC0.pin.AD0.Rx_idx=126;MCHP.module.AFEC0.pin.AD0.ABCD=-2;MCHP.module.AFEC0.pin.AD1.txt={ 'PA21'};MCHP.module.AFEC0.pin.AD1.Rx_idx=21;MCHP.module.AFEC0.pin.AD1.ABCD=-2;MCHP.module.AFEC0.pin.AD2.txt={ 'PB3'};MCHP.module.AFEC0.pin.AD2.Rx_idx=35;MCHP.module.AFEC0.pin.AD2.ABCD=-2;MCHP.module.AFEC0.pin.AD3.txt={ 'PE5'};MCHP.module.AFEC0.pin.AD3.Rx_idx=133;MCHP.module.AFEC0.pin.AD3.ABCD=-2;MCHP.module.AFEC0.pin.AD4.txt={ 'PE4'};MCHP.module.AFEC0.pin.AD4.Rx_idx=132;MCHP.module.AFEC0.pin.AD4.ABCD=-2;MCHP.module.AFEC0.pin.AD5.txt={ 'PB2'};MCHP.module.AFEC0.pin.AD5.Rx_idx=34;MCHP.module.AFEC0.pin.AD5.ABCD=-2;MCHP.module.AFEC0.pin.AD6.txt={ 'PA17'};MCHP.module.AFEC0.pin.AD6.Rx_idx=17;MCHP.module.AFEC0.pin.AD6.ABCD=-2;MCHP.module.AFEC0.pin.AD7.txt={ 'PA18'};MCHP.module.AFEC0.pin.AD7.Rx_idx=18;MCHP.module.AFEC0.pin.AD7.ABCD=-2;MCHP.module.AFEC0.pin.AD8.txt={ 'PA19'};MCHP.module.AFEC0.pin.AD8.Rx_idx=19;MCHP.module.AFEC0.pin.AD8.ABCD=-2;MCHP.module.AFEC0.pin.AD9.txt={ 'PA20'};MCHP.module.AFEC0.pin.AD9.Rx_idx=20;MCHP.module.AFEC0.pin.AD9.ABCD=-2;MCHP.module.AFEC0.pin.AD10.txt={ 'PB0'};MCHP.module.AFEC0.pin.AD10.Rx_idx=32;MCHP.module.AFEC0.pin.AD10.ABCD=-2;MCHP.module.DACC.PID=30;MCHP.module.DACC.vector='DACC';MCHP.module.DACC.pin.DAC0.txt={ 'PB13'};MCHP.module.DACC.pin.DAC0.Rx_idx=45;MCHP.module.DACC.pin.DAC0.ABCD=-2;MCHP.module.DACC.pin.DAC1.txt={ 'PD0'};MCHP.module.DACC.pin.DAC1.Rx_idx=96;MCHP.module.DACC.pin.DAC1.ABCD=-2;MCHP.module.DACC.pin.DATRG.txt={ 'PA2'};MCHP.module.DACC.pin.DATRG.Rx_idx=2;MCHP.module.DACC.pin.DATRG.ABCD=2;MCHP.module.PWM0.PID=31;MCHP.module.PWM0.vector='PWM0';MCHP.module.PWM0.pin.PWMEXTRG0.txt={ 'PA10'};MCHP.module.PWM0.pin.PWMEXTRG0.Rx_idx=10;MCHP.module.PWM0.pin.PWMEXTRG0.ABCD=1;MCHP.module.PWM0.pin.PWMEXTRG1.txt={ 'PA22'};MCHP.module.PWM0.pin.PWMEXTRG1.Rx_idx=22;MCHP.module.PWM0.pin.PWMEXTRG1.ABCD=1;MCHP.module.PWM0.pin.PWMFI0.txt={ 'PA9'};MCHP.module.PWM0.pin.PWMFI0.Rx_idx=9;MCHP.module.PWM0.pin.PWMFI0.ABCD=2;MCHP.module.PWM0.pin.PWMFI1.txt={ 'PD8'};MCHP.module.PWM0.pin.PWMFI1.Rx_idx=104;MCHP.module.PWM0.pin.PWMFI1.ABCD=1;MCHP.module.PWM0.pin.PWMFI2.txt={ 'PD9'};MCHP.module.PWM0.pin.PWMFI2.Rx_idx=105;MCHP.module.PWM0.pin.PWMFI2.ABCD=1;MCHP.module.PWM0.pin.PWMH0.txt=reshape({ 'PA0','PA11','PA23','PB0','PD11','PD20'},1,6);MCHP.module.PWM0.pin.PWMH0.Rx_idx=reshape([0 11 23 32 107 116],1,6);MCHP.module.PWM0.pin.PWMH0.ABCD=reshape([0 1 1 0 1 0],1,6);MCHP.module.PWM0.pin.PWMH1.txt=reshape({ 'PA2','PA12','PA24','PB1','PD21'},1,5);MCHP.module.PWM0.pin.PWMH1.Rx_idx=reshape([2 12 24 33 117],1,5);MCHP.module.PWM0.pin.PWMH1.ABCD=reshape([0 1 1 0 0],1,5);MCHP.module.PWM0.pin.PWMH2.txt=reshape({ 'PA13','PA25','PB4','PC19','PD22'},1,5);MCHP.module.PWM0.pin.PWMH2.Rx_idx=reshape([13 25 36 83 118],1,5);MCHP.module.PWM0.pin.PWMH2.ABCD=reshape([1 1 1 1 0],1,5);MCHP.module.PWM0.pin.PWMH3.txt=reshape({ 'PA7','PA14','PA17','PC13','PC21','PD23'},1,6);MCHP.module.PWM0.pin.PWMH3.Rx_idx=reshape([7 14 17 77 85 119],1,6);MCHP.module.PWM0.pin.PWMH3.ABCD=reshape([1 1 2 1 1 0],1,6);MCHP.module.PWM0.pin.PWML0.txt=reshape({ 'PA1','PA19','PB5','PC0','PD10','PD24'},1,6);MCHP.module.PWM0.pin.PWML0.Rx_idx=reshape([1 19 37 64 106 120],1,6);MCHP.module.PWM0.pin.PWML0.ABCD=reshape([0 1 1 1 1 0],1,6);MCHP.module.PWM0.pin.PWML1.txt=reshape({ 'PA20','PB12','PC1','PC18','PD25'},1,5);MCHP.module.PWM0.pin.PWML1.Rx_idx=reshape([20 44 65 82 121],1,5);MCHP.module.PWM0.pin.PWML1.ABCD=reshape([1 0 1 1 0],1,5);MCHP.module.PWM0.pin.PWML2.txt=reshape({ 'PA16','PA30','PB13','PC2','PC20','PD26'},1,6);MCHP.module.PWM0.pin.PWML2.Rx_idx=reshape([16 30 45 66 84 122],1,6);MCHP.module.PWM0.pin.PWML2.ABCD=reshape([2 0 0 1 1 0],1,6);MCHP.module.PWM0.pin.PWML3.txt=reshape({ 'PA15','PC3','PC15','PC22','PD27'},1,5);MCHP.module.PWM0.pin.PWML3.Rx_idx=reshape([15 67 79 86 123],1,5);MCHP.module.PWM0.pin.PWML3.ABCD=reshape([2 1 1 1 0],1,5);MCHP.module.ICM.PID=32;MCHP.module.ICM.vector='ICM';MCHP.module.ACC.PID=33;MCHP.module.ACC.vector='ACC';MCHP.module.USBHS.PID=34;MCHP.module.USBHS.vector='USBHS';MCHP.module.MCAN0(1).PID=35;MCHP.module.MCAN0(1).vector='MCAN0_INT0';MCHP.module.MCAN0(1).pin.CANRX0.txt={ 'PB3'};MCHP.module.MCAN0(1).pin.CANRX0.Rx_idx=35;MCHP.module.MCAN0(1).pin.CANRX0.ABCD=0;MCHP.module.MCAN0(1).pin.CANTX0.txt={ 'PB2'};MCHP.module.MCAN0(1).pin.CANTX0.Rx_idx=34;MCHP.module.MCAN0(1).pin.CANTX0.ABCD=0;MCHP.module.MCAN0(2).PID=36;MCHP.module.MCAN0(2).vector='MCAN0_INT1';MCHP.module.MCAN0(2).pin=reshape(MCHP_Fun.Hex2num('[]'),0,0);MCHP.module.MCAN1(1).PID=37;MCHP.module.MCAN1(1).vector='MCAN1_INT0';MCHP.module.MCAN1(1).pin.CANRX1.txt={ 'PC12'};MCHP.module.MCAN1(1).pin.CANRX1.Rx_idx=76;MCHP.module.MCAN1(1).pin.CANRX1.ABCD=2;MCHP.module.MCAN1(1).pin.CANTX1.txt=reshape({ 'PC14','PD12'},1,2);MCHP.module.MCAN1(1).pin.CANTX1.Rx_idx=reshape([78 108],1,2);MCHP.module.MCAN1(1).pin.CANTX1.ABCD=reshape([2 1],1,2);MCHP.module.MCAN1(2).PID=38;MCHP.module.MCAN1(2).vector='MCAN1_INT1';MCHP.module.MCAN1(2).pin=reshape(MCHP_Fun.Hex2num('[]'),0,0);MCHP.module.GMAC(1).PID=39;MCHP.module.GMAC(1).vector='GMAC';MCHP.module.GMAC(1).pin.GCOL.txt={ 'PD13'};MCHP.module.GMAC(1).pin.GCOL.Rx_idx=109;MCHP.module.GMAC(1).pin.GCOL.ABCD=0;MCHP.module.GMAC(1).pin.GCRS.txt={ 'PD10'};MCHP.module.GMAC(1).pin.GCRS.Rx_idx=106;MCHP.module.GMAC(1).pin.GCRS.ABCD=0;MCHP.module.GMAC(1).pin.GMDC.txt={ 'PD8'};MCHP.module.GMAC(1).pin.GMDC.Rx_idx=104;MCHP.module.GMAC(1).pin.GMDC.ABCD=0;MCHP.module.GMAC(1).pin.GMDIO.txt={ 'PD9'};MCHP.module.GMAC(1).pin.GMDIO.Rx_idx=105;MCHP.module.GMAC(1).pin.GMDIO.ABCD=0;MCHP.module.GMAC(1).pin.GRXCK.txt={ 'PD14'};MCHP.module.GMAC(1).pin.GRXCK.Rx_idx=110;MCHP.module.GMAC(1).pin.GRXCK.ABCD=0;MCHP.module.GMAC(1).pin.GRXDV.txt={ 'PD4'};MCHP.module.GMAC(1).pin.GRXDV.Rx_idx=100;MCHP.module.GMAC(1).pin.GRXDV.ABCD=0;MCHP.module.GMAC(1).pin.GRXER.txt={ 'PD7'};MCHP.module.GMAC(1).pin.GRXER.Rx_idx=103;MCHP.module.GMAC(1).pin.GRXER.ABCD=0;MCHP.module.GMAC(1).pin.GRX0.txt={ 'PD5'};MCHP.module.GMAC(1).pin.GRX0.Rx_idx=101;MCHP.module.GMAC(1).pin.GRX0.ABCD=0;MCHP.module.GMAC(1).pin.GRX1.txt={ 'PD6'};MCHP.module.GMAC(1).pin.GRX1.Rx_idx=102;MCHP.module.GMAC(1).pin.GRX1.ABCD=0;MCHP.module.GMAC(1).pin.GRX2.txt={ 'PD11'};MCHP.module.GMAC(1).pin.GRX2.Rx_idx=107;MCHP.module.GMAC(1).pin.GRX2.ABCD=0;MCHP.module.GMAC(1).pin.GRX3.txt={ 'PD12'};MCHP.module.GMAC(1).pin.GRX3.Rx_idx=108;MCHP.module.GMAC(1).pin.GRX3.ABCD=0;MCHP.module.GMAC(1).pin.GTSUCOMP.txt=reshape({ 'PB1','PB12','PD11','PD20'},1,4);MCHP.module.GMAC(1).pin.GTSUCOMP.Rx_idx=reshape([33 44 107 116],1,4);MCHP.module.GMAC(1).pin.GTSUCOMP.ABCD=reshape([1 1 2 2],1,4);MCHP.module.GMAC(1).pin.GTXCK.txt={ 'PD0'};MCHP.module.GMAC(1).pin.GTXCK.Rx_idx=96;MCHP.module.GMAC(1).pin.GTXCK.ABCD=0;MCHP.module.GMAC(1).pin.GTXEN.txt={ 'PD1'};MCHP.module.GMAC(1).pin.GTXEN.Rx_idx=97;MCHP.module.GMAC(1).pin.GTXEN.ABCD=0;MCHP.module.GMAC(1).pin.GTXER.txt={ 'PD17'};MCHP.module.GMAC(1).pin.GTXER.Rx_idx=113;MCHP.module.GMAC(1).pin.GTXER.ABCD=0;MCHP.module.GMAC(1).pin.GTX0.txt={ 'PD2'};MCHP.module.GMAC(1).pin.GTX0.Rx_idx=98;MCHP.module.GMAC(1).pin.GTX0.ABCD=0;MCHP.module.GMAC(1).pin.GTX1.txt={ 'PD3'};MCHP.module.GMAC(1).pin.GTX1.Rx_idx=99;MCHP.module.GMAC(1).pin.GTX1.ABCD=0;MCHP.module.GMAC(1).pin.GTX2.txt={ 'PD15'};MCHP.module.GMAC(1).pin.GTX2.Rx_idx=111;MCHP.module.GMAC(1).pin.GTX2.ABCD=0;MCHP.module.GMAC(1).pin.GTX3.txt={ 'PD16'};MCHP.module.GMAC(1).pin.GTX3.Rx_idx=112;MCHP.module.GMAC(1).pin.GTX3.ABCD=0;MCHP.module.GMAC(2).PID=66;MCHP.module.GMAC(2).vector='GMAC_Q1';MCHP.module.GMAC(2).pin=reshape(MCHP_Fun.Hex2num('[]'),0,0);MCHP.module.GMAC(3).PID=67;MCHP.module.GMAC(3).vector='GMAC_Q2';MCHP.module.GMAC(3).pin=reshape(MCHP_Fun.Hex2num('[]'),0,0);MCHP.module.GMAC(4).PID=71;MCHP.module.GMAC(4).vector='GMAC_Q3';MCHP.module.GMAC(4).pin=reshape(MCHP_Fun.Hex2num('[]'),0,0);MCHP.module.GMAC(5).PID=72;MCHP.module.GMAC(5).vector='GMAC_Q4';MCHP.module.GMAC(5).pin=reshape(MCHP_Fun.Hex2num('[]'),0,0);MCHP.module.GMAC(6).PID=73;MCHP.module.GMAC(6).vector='GMAC_Q5';MCHP.module.GMAC(6).pin=reshape(MCHP_Fun.Hex2num('[]'),0,0);MCHP.module.AFEC1.PID=40;MCHP.module.AFEC1.vector='AFEC1';MCHP.module.AFEC1.pin.ADTRG.txt={ 'PD9'};MCHP.module.AFEC1.pin.ADTRG.Rx_idx=105;MCHP.module.AFEC1.pin.ADTRG.ABCD=2;MCHP.module.AFEC1.pin.AD0.txt={ 'PB1'};MCHP.module.AFEC1.pin.AD0.Rx_idx=33;MCHP.module.AFEC1.pin.AD0.ABCD=-2;MCHP.module.AFEC1.pin.AD1.txt={ 'PC13'};MCHP.module.AFEC1.pin.AD1.Rx_idx=77;MCHP.module.AFEC1.pin.AD1.ABCD=-2;MCHP.module.AFEC1.pin.AD2.txt={ 'PC15'};MCHP.module.AFEC1.pin.AD2.Rx_idx=79;MCHP.module.AFEC1.pin.AD2.ABCD=-2;MCHP.module.AFEC1.pin.AD3.txt={ 'PC12'};MCHP.module.AFEC1.pin.AD3.Rx_idx=76;MCHP.module.AFEC1.pin.AD3.ABCD=-2;MCHP.module.AFEC1.pin.AD4.txt={ 'PC29'};MCHP.module.AFEC1.pin.AD4.Rx_idx=93;MCHP.module.AFEC1.pin.AD4.ABCD=-2;MCHP.module.AFEC1.pin.AD5.txt={ 'PC30'};MCHP.module.AFEC1.pin.AD5.Rx_idx=94;MCHP.module.AFEC1.pin.AD5.ABCD=-2;MCHP.module.AFEC1.pin.AD6.txt={ 'PC31'};MCHP.module.AFEC1.pin.AD6.Rx_idx=95;MCHP.module.AFEC1.pin.AD6.ABCD=-2;MCHP.module.AFEC1.pin.AD7.txt={ 'PC26'};MCHP.module.AFEC1.pin.AD7.Rx_idx=90;MCHP.module.AFEC1.pin.AD7.ABCD=-2;MCHP.module.AFEC1.pin.AD8.txt={ 'PC27'};MCHP.module.AFEC1.pin.AD8.Rx_idx=91;MCHP.module.AFEC1.pin.AD8.ABCD=-2;MCHP.module.AFEC1.pin.AD9.txt={ 'PC0'};MCHP.module.AFEC1.pin.AD9.Rx_idx=64;MCHP.module.AFEC1.pin.AD9.ABCD=-2;MCHP.module.AFEC1.pin.AD10.txt={ 'PE3'};MCHP.module.AFEC1.pin.AD10.Rx_idx=131;MCHP.module.AFEC1.pin.AD10.ABCD=-2;MCHP.module.AFEC1.pin.AD11.txt={ 'PE0'};MCHP.module.AFEC1.pin.AD11.Rx_idx=128;MCHP.module.AFEC1.pin.AD11.ABCD=-2;MCHP.module.TWIHS2.PID=41;MCHP.module.TWIHS2.vector='TWIHS2';MCHP.module.TWIHS2.pin.TWCK2.txt={ 'PD28'};MCHP.module.TWIHS2.pin.TWCK2.Rx_idx=124;MCHP.module.TWIHS2.pin.TWCK2.ABCD=2;MCHP.module.TWIHS2.pin.TWD2.txt={ 'PD27'};MCHP.module.TWIHS2.pin.TWD2.Rx_idx=123;MCHP.module.TWIHS2.pin.TWD2.ABCD=2;MCHP.module.SPI1.PID=42;MCHP.module.SPI1.vector='SPI1';MCHP.module.SPI1.pin.MISO.txt={ 'PC26'};MCHP.module.SPI1.pin.MISO.Rx_idx=90;MCHP.module.SPI1.pin.MISO.ABCD=2;MCHP.module.SPI1.pin.MOSI.txt={ 'PC27'};MCHP.module.SPI1.pin.MOSI.Rx_idx=91;MCHP.module.SPI1.pin.MOSI.ABCD=2;MCHP.module.SPI1.pin.NPCS0.txt={ 'PC25'};MCHP.module.SPI1.pin.NPCS0.Rx_idx=89;MCHP.module.SPI1.pin.NPCS0.ABCD=2;MCHP.module.SPI1.pin.NPCS1.txt=reshape({ 'PC28','PD0'},1,2);MCHP.module.SPI1.pin.NPCS1.Rx_idx=reshape([92 96],1,2);MCHP.module.SPI1.pin.NPCS1.ABCD=reshape([2 2],1,2);MCHP.module.SPI1.pin.NPCS2.txt=reshape({ 'PC29','PD1'},1,2);MCHP.module.SPI1.pin.NPCS2.Rx_idx=reshape([93 97],1,2);MCHP.module.SPI1.pin.NPCS2.ABCD=reshape([2 2],1,2);MCHP.module.SPI1.pin.NPCS3.txt=reshape({ 'PC30','PD2'},1,2);MCHP.module.SPI1.pin.NPCS3.Rx_idx=reshape([94 98],1,2);MCHP.module.SPI1.pin.NPCS3.ABCD=reshape([2 2],1,2);MCHP.module.SPI1.pin.SPCK.txt={ 'PC24'};MCHP.module.SPI1.pin.SPCK.Rx_idx=88;MCHP.module.SPI1.pin.SPCK.ABCD=2;MCHP.module.QSPI.PID=43;MCHP.module.QSPI.vector='QSPI';MCHP.module.QSPI.pin.QCS.txt={ 'PA11'};MCHP.module.QSPI.pin.QCS.Rx_idx=11;MCHP.module.QSPI.pin.QCS.ABCD=0;MCHP.module.QSPI.pin.QIO0.txt={ 'PA13'};MCHP.module.QSPI.pin.QIO0.Rx_idx=13;MCHP.module.QSPI.pin.QIO0.ABCD=0;MCHP.module.QSPI.pin.QIO1.txt={ 'PA12'};MCHP.module.QSPI.pin.QIO1.Rx_idx=12;MCHP.module.QSPI.pin.QIO1.ABCD=0;MCHP.module.QSPI.pin.QIO2.txt={ 'PA17'};MCHP.module.QSPI.pin.QIO2.Rx_idx=17;MCHP.module.QSPI.pin.QIO2.ABCD=0;MCHP.module.QSPI.pin.QIO3.txt={ 'PD31'};MCHP.module.QSPI.pin.QIO3.Rx_idx=127;MCHP.module.QSPI.pin.QIO3.ABCD=0;MCHP.module.QSPI.pin.QSCK.txt={ 'PA14'};MCHP.module.QSPI.pin.QSCK.Rx_idx=14;MCHP.module.QSPI.pin.QSCK.ABCD=0;MCHP.module.UART2.PID=44;MCHP.module.UART2.vector='UART2';MCHP.module.UART2.pin.URXD2.txt={ 'PD25'};MCHP.module.UART2.pin.URXD2.Rx_idx=121;MCHP.module.UART2.pin.URXD2.ABCD=2;MCHP.module.UART2.pin.UTXD2.txt={ 'PD26'};MCHP.module.UART2.pin.UTXD2.Rx_idx=122;MCHP.module.UART2.pin.UTXD2.ABCD=2;MCHP.module.UART3.PID=45;MCHP.module.UART3.vector='UART3';MCHP.module.UART3.pin.URXD3.txt={ 'PD28'};MCHP.module.UART3.pin.URXD3.Rx_idx=124;MCHP.module.UART3.pin.URXD3.ABCD=0;MCHP.module.UART3.pin.UTXD3.txt=reshape({ 'PD30','PD31'},1,2);MCHP.module.UART3.pin.UTXD3.Rx_idx=reshape([126 127],1,2);MCHP.module.UART3.pin.UTXD3.ABCD=reshape([0 1],1,2);MCHP.module.UART4.PID=46;MCHP.module.UART4.vector='UART4';MCHP.module.UART4.pin.URXD4.txt={ 'PD18'};MCHP.module.UART4.pin.URXD4.Rx_idx=114;MCHP.module.UART4.pin.URXD4.ABCD=2;MCHP.module.UART4.pin.UTXD4.txt=reshape({ 'PD3','PD19'},1,2);MCHP.module.UART4.pin.UTXD4.Rx_idx=reshape([99 115],1,2);MCHP.module.UART4.pin.UTXD4.ABCD=reshape([2 2],1,2);MCHP.module.TC2(1).PID=47;MCHP.module.TC2(1).vector='TC6';MCHP.module.TC2(1).pin.TCLK6.txt={ 'PC7'};MCHP.module.TC2(1).pin.TCLK6.Rx_idx=71;MCHP.module.TC2(1).pin.TCLK6.ABCD=1;MCHP.module.TC2(1).pin.TCLK7.txt={ 'PC10'};MCHP.module.TC2(1).pin.TCLK7.Rx_idx=74;MCHP.module.TC2(1).pin.TCLK7.ABCD=1;MCHP.module.TC2(1).pin.TCLK8.txt={ 'PC14'};MCHP.module.TC2(1).pin.TCLK8.Rx_idx=78;MCHP.module.TC2(1).pin.TCLK8.ABCD=1;MCHP.module.TC2(1).pin.TIOA6.txt={ 'PC5'};MCHP.module.TC2(1).pin.TIOA6.Rx_idx=69;MCHP.module.TC2(1).pin.TIOA6.ABCD=1;MCHP.module.TC2(1).pin.TIOA7.txt={ 'PC8'};MCHP.module.TC2(1).pin.TIOA7.Rx_idx=72;MCHP.module.TC2(1).pin.TIOA7.ABCD=1;MCHP.module.TC2(1).pin.TIOA8.txt={ 'PC11'};MCHP.module.TC2(1).pin.TIOA8.Rx_idx=75;MCHP.module.TC2(1).pin.TIOA8.ABCD=1;MCHP.module.TC2(1).pin.TIOB6.txt={ 'PC6'};MCHP.module.TC2(1).pin.TIOB6.Rx_idx=70;MCHP.module.TC2(1).pin.TIOB6.ABCD=1;MCHP.module.TC2(1).pin.TIOB7.txt={ 'PC9'};MCHP.module.TC2(1).pin.TIOB7.Rx_idx=73;MCHP.module.TC2(1).pin.TIOB7.ABCD=1;MCHP.module.TC2(1).pin.TIOB8.txt={ 'PC12'};MCHP.module.TC2(1).pin.TIOB8.Rx_idx=76;MCHP.module.TC2(1).pin.TIOB8.ABCD=1;MCHP.module.TC2(2).PID=48;MCHP.module.TC2(2).vector='TC7';MCHP.module.TC2(2).pin=reshape(MCHP_Fun.Hex2num('[]'),0,0);MCHP.module.TC2(3).PID=49;MCHP.module.TC2(3).vector='TC8';MCHP.module.TC2(3).pin=reshape(MCHP_Fun.Hex2num('[]'),0,0);MCHP.module.TC3(1).PID=50;MCHP.module.TC3(1).vector='TC9';MCHP.module.TC3(1).pin.TCLK9.txt={ 'PE2'};MCHP.module.TC3(1).pin.TCLK9.Rx_idx=130;MCHP.module.TC3(1).pin.TCLK9.ABCD=1;MCHP.module.TC3(1).pin.TCLK10.txt={ 'PE5'};MCHP.module.TC3(1).pin.TCLK10.Rx_idx=133;MCHP.module.TC3(1).pin.TCLK10.ABCD=1;MCHP.module.TC3(1).pin.TCLK11.txt={ 'PD24'};MCHP.module.TC3(1).pin.TCLK11.Rx_idx=120;MCHP.module.TC3(1).pin.TCLK11.ABCD=2;MCHP.module.TC3(1).pin.TIOA9.txt={ 'PE0'};MCHP.module.TC3(1).pin.TIOA9.Rx_idx=128;MCHP.module.TC3(1).pin.TIOA9.ABCD=1;MCHP.module.TC3(1).pin.TIOA10.txt={ 'PE3'};MCHP.module.TC3(1).pin.TIOA10.Rx_idx=131;MCHP.module.TC3(1).pin.TIOA10.ABCD=1;MCHP.module.TC3(1).pin.TIOA11.txt={ 'PD21'};MCHP.module.TC3(1).pin.TIOA11.Rx_idx=117;MCHP.module.TC3(1).pin.TIOA11.ABCD=2;MCHP.module.TC3(1).pin.TIOB9.txt={ 'PE1'};MCHP.module.TC3(1).pin.TIOB9.Rx_idx=129;MCHP.module.TC3(1).pin.TIOB9.ABCD=1;MCHP.module.TC3(1).pin.TIOB10.txt={ 'PE4'};MCHP.module.TC3(1).pin.TIOB10.Rx_idx=132;MCHP.module.TC3(1).pin.TIOB10.ABCD=1;MCHP.module.TC3(1).pin.TIOB11.txt={ 'PD22'};MCHP.module.TC3(1).pin.TIOB11.Rx_idx=118;MCHP.module.TC3(1).pin.TIOB11.ABCD=2;MCHP.module.TC3(2).PID=51;MCHP.module.TC3(2).vector='TC10';MCHP.module.TC3(2).pin=reshape(MCHP_Fun.Hex2num('[]'),0,0);MCHP.module.TC3(3).PID=52;MCHP.module.TC3(3).vector='TC11';MCHP.module.TC3(3).pin=reshape(MCHP_Fun.Hex2num('[]'),0,0);MCHP.module.AES.PID=56;MCHP.module.AES.vector='AES';MCHP.module.TRNG.PID=57;MCHP.module.TRNG.vector='TRNG';MCHP.module.XDMAC.PID=58;MCHP.module.XDMAC.vector='XDMAC';MCHP.module.ISI.PID=59;MCHP.module.ISI.vector='ISI';MCHP.module.ISI.pin.D0.txt={ 'PD22'};MCHP.module.ISI.pin.D0.Rx_idx=118;MCHP.module.ISI.pin.D0.ABCD=3;MCHP.module.ISI.pin.D1.txt={ 'PD21'};MCHP.module.ISI.pin.D1.Rx_idx=117;MCHP.module.ISI.pin.D1.ABCD=3;MCHP.module.ISI.pin.D2.txt={ 'PB3'};MCHP.module.ISI.pin.D2.Rx_idx=35;MCHP.module.ISI.pin.D2.ABCD=3;MCHP.module.ISI.pin.D3.txt={ 'PA9'};MCHP.module.ISI.pin.D3.Rx_idx=9;MCHP.module.ISI.pin.D3.ABCD=1;MCHP.module.ISI.pin.D4.txt={ 'PA5'};MCHP.module.ISI.pin.D4.Rx_idx=5;MCHP.module.ISI.pin.D4.ABCD=1;MCHP.module.ISI.pin.D5.txt={ 'PD11'};MCHP.module.ISI.pin.D5.Rx_idx=107;MCHP.module.ISI.pin.D5.ABCD=3;MCHP.module.ISI.pin.D6.txt={ 'PD12'};MCHP.module.ISI.pin.D6.Rx_idx=108;MCHP.module.ISI.pin.D6.ABCD=3;MCHP.module.ISI.pin.D7.txt={ 'PA27'};MCHP.module.ISI.pin.D7.Rx_idx=27;MCHP.module.ISI.pin.D7.ABCD=3;MCHP.module.ISI.pin.D8.txt={ 'PD27'};MCHP.module.ISI.pin.D8.Rx_idx=123;MCHP.module.ISI.pin.D8.ABCD=3;MCHP.module.ISI.pin.D9.txt={ 'PD28'};MCHP.module.ISI.pin.D9.Rx_idx=124;MCHP.module.ISI.pin.D9.ABCD=3;MCHP.module.ISI.pin.D10.txt={ 'PD30'};MCHP.module.ISI.pin.D10.Rx_idx=126;MCHP.module.ISI.pin.D10.ABCD=3;MCHP.module.ISI.pin.D11.txt={ 'PD31'};MCHP.module.ISI.pin.D11.Rx_idx=127;MCHP.module.ISI.pin.D11.ABCD=3;MCHP.module.ISI.pin.HSYNC.txt={ 'PD24'};MCHP.module.ISI.pin.HSYNC.Rx_idx=120;MCHP.module.ISI.pin.HSYNC.ABCD=3;MCHP.module.ISI.pin.PCK.txt={ 'PA24'};MCHP.module.ISI.pin.PCK.Rx_idx=24;MCHP.module.ISI.pin.PCK.ABCD=3;MCHP.module.ISI.pin.VSYNC.txt={ 'PD25'};MCHP.module.ISI.pin.VSYNC.Rx_idx=121;MCHP.module.ISI.pin.VSYNC.ABCD=3;MCHP.module.PWM1.PID=60;MCHP.module.PWM1.vector='PWM1';MCHP.module.PWM1.pin.PWMEXTRG0.txt={ 'PA30'};MCHP.module.PWM1.pin.PWMEXTRG0.Rx_idx=30;MCHP.module.PWM1.pin.PWMEXTRG0.ABCD=1;MCHP.module.PWM1.pin.PWMEXTRG1.txt={ 'PA18'};MCHP.module.PWM1.pin.PWMEXTRG1.Rx_idx=18;MCHP.module.PWM1.pin.PWMEXTRG1.ABCD=0;MCHP.module.PWM1.pin.PWMFI0.txt={ 'PA21'};MCHP.module.PWM1.pin.PWMFI0.Rx_idx=21;MCHP.module.PWM1.pin.PWMFI0.ABCD=2;MCHP.module.PWM1.pin.PWMFI1.txt={ 'PA26'};MCHP.module.PWM1.pin.PWMFI1.Rx_idx=26;MCHP.module.PWM1.pin.PWMFI1.ABCD=3;MCHP.module.PWM1.pin.PWMFI2.txt={ 'PA28'};MCHP.module.PWM1.pin.PWMFI2.Rx_idx=28;MCHP.module.PWM1.pin.PWMFI2.ABCD=3;MCHP.module.PWM1.pin.PWMH0.txt=reshape({ 'PA12','PD1'},1,2);MCHP.module.PWM1.pin.PWMH0.Rx_idx=reshape([12 97],1,2);MCHP.module.PWM1.pin.PWMH0.ABCD=reshape([2 1],1,2);MCHP.module.PWM1.pin.PWMH1.txt=reshape({ 'PA14','PD3'},1,2);MCHP.module.PWM1.pin.PWMH1.Rx_idx=reshape([14 99],1,2);MCHP.module.PWM1.pin.PWMH1.ABCD=reshape([2 1],1,2);MCHP.module.PWM1.pin.PWMH2.txt=reshape({ 'PA31','PD5'},1,2);MCHP.module.PWM1.pin.PWMH2.Rx_idx=reshape([31 101],1,2);MCHP.module.PWM1.pin.PWMH2.ABCD=reshape([3 1],1,2);MCHP.module.PWM1.pin.PWMH3.txt=reshape({ 'PA8','PD7'},1,2);MCHP.module.PWM1.pin.PWMH3.Rx_idx=reshape([8 103],1,2);MCHP.module.PWM1.pin.PWMH3.ABCD=reshape([0 1],1,2);MCHP.module.PWM1.pin.PWML0.txt=reshape({ 'PA11','PD0'},1,2);MCHP.module.PWM1.pin.PWML0.Rx_idx=reshape([11 96],1,2);MCHP.module.PWM1.pin.PWML0.ABCD=reshape([2 1],1,2);MCHP.module.PWM1.pin.PWML1.txt=reshape({ 'PA13','PD2'},1,2);MCHP.module.PWM1.pin.PWML1.Rx_idx=reshape([13 98],1,2);MCHP.module.PWM1.pin.PWML1.ABCD=reshape([2 1],1,2);MCHP.module.PWM1.pin.PWML2.txt=reshape({ 'PA23','PD4'},1,2);MCHP.module.PWM1.pin.PWML2.Rx_idx=reshape([23 100],1,2);MCHP.module.PWM1.pin.PWML2.ABCD=reshape([3 1],1,2);MCHP.module.PWM1.pin.PWML3.txt=reshape({ 'PA5','PD6'},1,2);MCHP.module.PWM1.pin.PWML3.Rx_idx=reshape([5 102],1,2);MCHP.module.PWM1.pin.PWML3.ABCD=reshape([0 1],1,2);MCHP.module.FPU(1).PID=61;MCHP.module.FPU(1).vector='FPU';MCHP.module.FPU(2).PID=68;MCHP.module.FPU(2).vector='IXC';MCHP.module.RSWDT.PID=63;MCHP.module.RSWDT.vector='RSWDT';MCHP.module.SCB(1).PID=64;MCHP.module.SCB(1).vector='CCW';MCHP.module.SCB(2).PID=65;MCHP.module.SCB(2).vector='CCF';MCHP.module.I2SC0.PID=69;MCHP.module.I2SC0.vector='I2SC0';MCHP.module.I2SC0.pin.CK.txt={ 'PA1'};MCHP.module.I2SC0.pin.CK.Rx_idx=1;MCHP.module.I2SC0.pin.CK.ABCD=3;MCHP.module.I2SC0.pin.DI0.txt={ 'PA16'};MCHP.module.I2SC0.pin.DI0.Rx_idx=16;MCHP.module.I2SC0.pin.DI0.ABCD=3;MCHP.module.I2SC0.pin.DO0.txt={ 'PA30'};MCHP.module.I2SC0.pin.DO0.Rx_idx=30;MCHP.module.I2SC0.pin.DO0.ABCD=3;MCHP.module.I2SC0.pin.MCK.txt={ 'PA0'};MCHP.module.I2SC0.pin.MCK.Rx_idx=0;MCHP.module.I2SC0.pin.MCK.ABCD=3;MCHP.module.I2SC0.pin.WS.txt={ 'PA15'};MCHP.module.I2SC0.pin.WS.Rx_idx=15;MCHP.module.I2SC0.pin.WS.ABCD=3;MCHP.module.I2SC1.PID=70;MCHP.module.I2SC1.vector='I2SC1';MCHP.module.I2SC1.pin.CK.txt={ 'PA20'};MCHP.module.I2SC1.pin.CK.Rx_idx=20;MCHP.module.I2SC1.pin.CK.ABCD=3;MCHP.module.I2SC1.pin.DI0.txt={ 'PE2'};MCHP.module.I2SC1.pin.DI0.Rx_idx=130;MCHP.module.I2SC1.pin.DI0.ABCD=2;MCHP.module.I2SC1.pin.DO0.txt={ 'PE1'};MCHP.module.I2SC1.pin.DO0.Rx_idx=129;MCHP.module.I2SC1.pin.DO0.ABCD=2;MCHP.module.I2SC1.pin.MCK.txt={ 'PA19'};MCHP.module.I2SC1.pin.MCK.Rx_idx=19;MCHP.module.I2SC1.pin.MCK.ABCD=3;MCHP.module.I2SC1.pin.WS.txt={ 'PE0'};MCHP.module.I2SC1.pin.WS.Rx_idx=128;MCHP.module.I2SC1.pin.WS.ABCD=2;MCHP.module.EBI.pin.A0.txt={ 'PC18'};MCHP.module.EBI.pin.A0.Rx_idx=82;MCHP.module.EBI.pin.A0.ABCD=0;MCHP.module.EBI.pin.A1.txt={ 'PC19'};MCHP.module.EBI.pin.A1.Rx_idx=83;MCHP.module.EBI.pin.A1.ABCD=0;MCHP.module.EBI.pin.A2.txt={ 'PC20'};MCHP.module.EBI.pin.A2.Rx_idx=84;MCHP.module.EBI.pin.A2.ABCD=0;MCHP.module.EBI.pin.A3.txt={ 'PC21'};MCHP.module.EBI.pin.A3.Rx_idx=85;MCHP.module.EBI.pin.A3.ABCD=0;MCHP.module.EBI.pin.A4.txt={ 'PC22'};MCHP.module.EBI.pin.A4.Rx_idx=86;MCHP.module.EBI.pin.A4.ABCD=0;MCHP.module.EBI.pin.A5.txt={ 'PC23'};MCHP.module.EBI.pin.A5.Rx_idx=87;MCHP.module.EBI.pin.A5.ABCD=0;MCHP.module.EBI.pin.A6.txt={ 'PC24'};MCHP.module.EBI.pin.A6.Rx_idx=88;MCHP.module.EBI.pin.A6.ABCD=0;MCHP.module.EBI.pin.A7.txt={ 'PC25'};MCHP.module.EBI.pin.A7.Rx_idx=89;MCHP.module.EBI.pin.A7.ABCD=0;MCHP.module.EBI.pin.A8.txt={ 'PC26'};MCHP.module.EBI.pin.A8.Rx_idx=90;MCHP.module.EBI.pin.A8.ABCD=0;MCHP.module.EBI.pin.A9.txt={ 'PC27'};MCHP.module.EBI.pin.A9.Rx_idx=91;MCHP.module.EBI.pin.A9.ABCD=0;MCHP.module.EBI.pin.A10.txt={ 'PC28'};MCHP.module.EBI.pin.A10.Rx_idx=92;MCHP.module.EBI.pin.A10.ABCD=0;MCHP.module.EBI.pin.A11.txt={ 'PC29'};MCHP.module.EBI.pin.A11.Rx_idx=93;MCHP.module.EBI.pin.A11.ABCD=0;MCHP.module.EBI.pin.A12.txt={ 'PC30'};MCHP.module.EBI.pin.A12.Rx_idx=94;MCHP.module.EBI.pin.A12.ABCD=0;MCHP.module.EBI.pin.A13.txt={ 'PC31'};MCHP.module.EBI.pin.A13.Rx_idx=95;MCHP.module.EBI.pin.A13.ABCD=0;MCHP.module.EBI.pin.A14.txt={ 'PA18'};MCHP.module.EBI.pin.A14.Rx_idx=18;MCHP.module.EBI.pin.A14.ABCD=2;MCHP.module.EBI.pin.A15.txt={ 'PA19'};MCHP.module.EBI.pin.A15.Rx_idx=19;MCHP.module.EBI.pin.A15.ABCD=2;MCHP.module.EBI.pin.A16.txt={ 'PA20'};MCHP.module.EBI.pin.A16.Rx_idx=20;MCHP.module.EBI.pin.A16.ABCD=2;MCHP.module.EBI.pin.A17.txt={ 'PA0'};MCHP.module.EBI.pin.A17.Rx_idx=0;MCHP.module.EBI.pin.A17.ABCD=2;MCHP.module.EBI.pin.A18.txt={ 'PA1'};MCHP.module.EBI.pin.A18.Rx_idx=1;MCHP.module.EBI.pin.A18.ABCD=2;MCHP.module.EBI.pin.A19.txt={ 'PA23'};MCHP.module.EBI.pin.A19.Rx_idx=23;MCHP.module.EBI.pin.A19.ABCD=2;MCHP.module.EBI.pin.A20.txt={ 'PA24'};MCHP.module.EBI.pin.A20.Rx_idx=24;MCHP.module.EBI.pin.A20.ABCD=2;MCHP.module.EBI.pin.A21.txt={ 'PC16'};MCHP.module.EBI.pin.A21.Rx_idx=80;MCHP.module.EBI.pin.A21.ABCD=0;MCHP.module.EBI.pin.A22.txt={ 'PC17'};MCHP.module.EBI.pin.A22.Rx_idx=81;MCHP.module.EBI.pin.A22.ABCD=0;MCHP.module.EBI.pin.A23.txt={ 'PA25'};MCHP.module.EBI.pin.A23.Rx_idx=25;MCHP.module.EBI.pin.A23.ABCD=2;MCHP.module.EBI.pin.D0.txt={ 'PC0'};MCHP.module.EBI.pin.D0.Rx_idx=64;MCHP.module.EBI.pin.D0.ABCD=0;MCHP.module.EBI.pin.D1.txt={ 'PC1'};MCHP.module.EBI.pin.D1.Rx_idx=65;MCHP.module.EBI.pin.D1.ABCD=0;MCHP.module.EBI.pin.D2.txt={ 'PC2'};MCHP.module.EBI.pin.D2.Rx_idx=66;MCHP.module.EBI.pin.D2.ABCD=0;MCHP.module.EBI.pin.D3.txt={ 'PC3'};MCHP.module.EBI.pin.D3.Rx_idx=67;MCHP.module.EBI.pin.D3.ABCD=0;MCHP.module.EBI.pin.D4.txt={ 'PC4'};MCHP.module.EBI.pin.D4.Rx_idx=68;MCHP.module.EBI.pin.D4.ABCD=0;MCHP.module.EBI.pin.D5.txt={ 'PC5'};MCHP.module.EBI.pin.D5.Rx_idx=69;MCHP.module.EBI.pin.D5.ABCD=0;MCHP.module.EBI.pin.D6.txt={ 'PC6'};MCHP.module.EBI.pin.D6.Rx_idx=70;MCHP.module.EBI.pin.D6.ABCD=0;MCHP.module.EBI.pin.D7.txt={ 'PC7'};MCHP.module.EBI.pin.D7.Rx_idx=71;MCHP.module.EBI.pin.D7.ABCD=0;MCHP.module.EBI.pin.D8.txt={ 'PE0'};MCHP.module.EBI.pin.D8.Rx_idx=128;MCHP.module.EBI.pin.D8.ABCD=0;MCHP.module.EBI.pin.D9.txt={ 'PE1'};MCHP.module.EBI.pin.D9.Rx_idx=129;MCHP.module.EBI.pin.D9.ABCD=0;MCHP.module.EBI.pin.D10.txt={ 'PE2'};MCHP.module.EBI.pin.D10.Rx_idx=130;MCHP.module.EBI.pin.D10.ABCD=0;MCHP.module.EBI.pin.D11.txt={ 'PE3'};MCHP.module.EBI.pin.D11.Rx_idx=131;MCHP.module.EBI.pin.D11.ABCD=0;MCHP.module.EBI.pin.D12.txt={ 'PE4'};MCHP.module.EBI.pin.D12.Rx_idx=132;MCHP.module.EBI.pin.D12.ABCD=0;MCHP.module.EBI.pin.D13.txt={ 'PE5'};MCHP.module.EBI.pin.D13.Rx_idx=133;MCHP.module.EBI.pin.D13.ABCD=0;MCHP.module.EBI.pin.D14.txt={ 'PA15'};MCHP.module.EBI.pin.D14.Rx_idx=15;MCHP.module.EBI.pin.D14.ABCD=0;MCHP.module.EBI.pin.D15.txt={ 'PA16'};MCHP.module.EBI.pin.D15.Rx_idx=16;MCHP.module.EBI.pin.D15.ABCD=0;MCHP.module.EBI.pin.NWAIT.txt={ 'PC13'};MCHP.module.EBI.pin.NWAIT.Rx_idx=77;MCHP.module.EBI.pin.NWAIT.ABCD=0;MCHP.module.EBI.pin.NCS0.txt={ 'PC14'};MCHP.module.EBI.pin.NCS0.Rx_idx=78;MCHP.module.EBI.pin.NCS0.ABCD=0;MCHP.module.EBI.pin.NCS1.txt=reshape({ 'PC15','PD18'},1,2);MCHP.module.EBI.pin.NCS1.Rx_idx=reshape([79 114],1,2);MCHP.module.EBI.pin.NCS1.ABCD=reshape([0 0],1,2);MCHP.module.EBI.pin.NCS2.txt={ 'PA22'};MCHP.module.EBI.pin.NCS2.Rx_idx=22;MCHP.module.EBI.pin.NCS2.ABCD=2;MCHP.module.EBI.pin.NCS3.txt=reshape({ 'PC12','PD19'},1,2);MCHP.module.EBI.pin.NCS3.Rx_idx=reshape([76 115],1,2);MCHP.module.EBI.pin.NCS3.ABCD=reshape([0 0],1,2);MCHP.module.EBI.pin.NWR0.txt={ 'PC8'};MCHP.module.EBI.pin.NWR0.Rx_idx=72;MCHP.module.EBI.pin.NWR0.ABCD=0;MCHP.module.EBI.pin.NWR1.txt={ 'PD15'};MCHP.module.EBI.pin.NWR1.Rx_idx=111;MCHP.module.EBI.pin.NWR1.ABCD=2;MCHP.module.EBI.pin.NRD.txt={ 'PC11'};MCHP.module.EBI.pin.NRD.Rx_idx=75;MCHP.module.EBI.pin.NRD.ABCD=0;MCHP.module.EBI.pin.NWE.txt={ 'PC8'};MCHP.module.EBI.pin.NWE.Rx_idx=72;MCHP.module.EBI.pin.NWE.ABCD=0;MCHP.module.EBI.pin.NBS0.txt={ 'PC18'};MCHP.module.EBI.pin.NBS0.Rx_idx=82;MCHP.module.EBI.pin.NBS0.ABCD=0;MCHP.module.EBI.pin.NBS1.txt={ 'PD15'};MCHP.module.EBI.pin.NBS1.Rx_idx=111;MCHP.module.EBI.pin.NBS1.ABCD=2;MCHP.module.EBI.pin.NANDALE.txt={ 'PC16'};MCHP.module.EBI.pin.NANDALE.Rx_idx=80;MCHP.module.EBI.pin.NANDALE.ABCD=0;MCHP.module.EBI.pin.NANDCLE.txt={ 'PC17'};MCHP.module.EBI.pin.NANDCLE.Rx_idx=81;MCHP.module.EBI.pin.NANDCLE.ABCD=0;MCHP.module.EBI.pin.NANDOE.txt={ 'PC9'};MCHP.module.EBI.pin.NANDOE.Rx_idx=73;MCHP.module.EBI.pin.NANDOE.ABCD=0;MCHP.module.EBI.pin.NANDWE.txt={ 'PC10'};MCHP.module.EBI.pin.NANDWE.Rx_idx=74;MCHP.module.EBI.pin.NANDWE.ABCD=0;MCHP.module.ICE.pin.TDI.txt={ 'PB4'};MCHP.module.ICE.pin.TDI.Rx_idx=36;MCHP.module.ICE.pin.TDI.ABCD=-2;MCHP.module.ICE.pin.TDO.txt={ 'PB5'};MCHP.module.ICE.pin.TDO.Rx_idx=37;MCHP.module.ICE.pin.TDO.ABCD=-2;MCHP.module.ICE.pin.TRACESWO.txt={ 'PB5'};MCHP.module.ICE.pin.TRACESWO.Rx_idx=37;MCHP.module.ICE.pin.TRACESWO.ABCD=-2;MCHP.module.ICE.pin.TMS.txt={ 'PB6'};MCHP.module.ICE.pin.TMS.Rx_idx=38;MCHP.module.ICE.pin.TMS.ABCD=-2;MCHP.module.ICE.pin.SWDIO.txt={ 'PB6'};MCHP.module.ICE.pin.SWDIO.Rx_idx=38;MCHP.module.ICE.pin.SWDIO.ABCD=-2;MCHP.module.ICE.pin.TCK.txt={ 'PB7'};MCHP.module.ICE.pin.TCK.Rx_idx=39;MCHP.module.ICE.pin.TCK.ABCD=-2;MCHP.module.ICE.pin.SWDCLK.txt={ 'PB7'};MCHP.module.ICE.pin.SWDCLK.Rx_idx=39;MCHP.module.ICE.pin.SWDCLK.ABCD=-2;MCHP.module.TPIU.pin.TRACECLK.txt={ 'PD8'};MCHP.module.TPIU.pin.TRACECLK.Rx_idx=104;MCHP.module.TPIU.pin.TRACECLK.ABCD=3;MCHP.module.TPIU.pin.TRACED0.txt={ 'PD4'};MCHP.module.TPIU.pin.TRACED0.Rx_idx=100;MCHP.module.TPIU.pin.TRACED0.ABCD=2;MCHP.module.TPIU.pin.TRACED1.txt={ 'PD5'};MCHP.module.TPIU.pin.TRACED1.Rx_idx=101;MCHP.module.TPIU.pin.TRACED1.ABCD=2;MCHP.module.TPIU.pin.TRACED2.txt={ 'PD6'};MCHP.module.TPIU.pin.TRACED2.Rx_idx=102;MCHP.module.TPIU.pin.TRACED2.ABCD=2;MCHP.module.TPIU.pin.TRACED3.txt={ 'PD7'};MCHP.module.TPIU.pin.TRACED3.Rx_idx=103;MCHP.module.TPIU.pin.TRACED3.ABCD=2;MCHP.module.FUSES.reglist={ 'GPNVMBITS'};MCHP.module.FUSES.reg.GPNVMBITS.caption='GPNVM Bits';MCHP.module.FUSES.reg.GPNVMBITS.bitfieldList=reshape({ 'SECURITY_BIT','BOOT_MODE','TCM_CONFIGURATION'},1,3);MCHP.module.FUSES.reg.GPNVMBITS.SECURITY_BIT.mask=2;MCHP.module.FUSES.reg.GPNVMBITS.SECURITY_BIT.choice=reshape({ 'CLEAR','SET'},1,2);MCHP.module.FUSES.reg.GPNVMBITS.SECURITY_BIT.choiceCaption=reshape({ 'clear','set'},1,2);MCHP.module.FUSES.reg.GPNVMBITS.SECURITY_BIT.choiceDefault='CLEAR';MCHP.module.FUSES.reg.GPNVMBITS.BOOT_MODE.mask=2;MCHP.module.FUSES.reg.GPNVMBITS.BOOT_MODE.choice=reshape({ 'CLEAR','SET'},1,2);MCHP.module.FUSES.reg.GPNVMBITS.BOOT_MODE.choiceCaption=reshape({ 'clear','set'},1,2);MCHP.module.FUSES.reg.GPNVMBITS.BOOT_MODE.choiceDefault='CLEAR';MCHP.module.FUSES.reg.GPNVMBITS.TCM_CONFIGURATION.mask=4;MCHP.module.FUSES.reg.GPNVMBITS.TCM_CONFIGURATION.choice=reshape({ '0','1','2','3','4'},1,5);MCHP.module.FUSES.reg.GPNVMBITS.TCM_CONFIGURATION.choiceCaption=reshape({ '0','1','2','3','4'},1,5);MCHP.module.FUSES.reg.GPNVMBITS.TCM_CONFIGURATION.choiceDefault='0x3';MCHP.modsrc.id_6490=1;MCHP.modsrc.id_6149=1;MCHP.modsrc.id_11147=2;MCHP.modsrc.id_6417=1;MCHP.modsrc.id_11246=1;MCHP.modsrc.id_EBI=1;MCHP.modsrc.id_6450=1;MCHP.modsrc.id_11046=1;MCHP.modsrc.id_6378=1;MCHP.modsrc.id_6449=1;MCHP.modsrc.id_11241=2;MCHP.modsrc.id_11105=1;MCHP.modsrc.id_6350=1;MCHP.modsrc.id_11282=1;MCHP.modsrc.id_11273=2;MCHP.modsrc.id_11004=5;MCHP.modsrc.id_44006=1;MCHP.modsrc.id_6343=2;MCHP.modsrc.id_11171=1;MCHP.modsrc.id_11009=1;MCHP.modsrc.id_11110=1;MCHP.modsrc.id_6056=1;MCHP.modsrc.id_6081=1;MCHP.modsrc.id_6498=1;MCHP.modsrc.id_6088=2;MCHP.modsrc.id_6078=1;MCHP.modsrc.id_6452=1;MCHP.modsrc.id_6082=4;MCHP.modsrc.id_6334=1;MCHP.modsrc.id_11210=3;MCHP.modsrc.id_6418=5;MCHP.modsrc.id_6089=3;MCHP.modsrc.id_11292=1;MCHP.modsrc.id_11300=1;MCHP.modsrc.id_6080=1;MCHP.modsrc.id_11161=1;MCHP.modsrc.id_1=1;MCHP.modsrc.id_SCnSCB=1;MCHP.modsrc.id_SCB=1;MCHP.modsrc.id_SysTick=1;MCHP.modsrc.id_NVIC=1;MCHP.modsrc.id_MPU=1;MCHP.modsrc.id_FPU=1;MCHP.modsrc.id_ICE=1;MCHP.modsrc.id_TPIU=1;MCHP.modsrc_id.id_6490.n=1;MCHP.modsrc_id.id_6490.name='ACC';MCHP.modsrc_id.id_6490.version='J';MCHP.modsrc_id.id_6149.n=1;MCHP.modsrc_id.id_6149.name='AES';MCHP.modsrc_id.id_6149.version='W';MCHP.modsrc_id.id_11147.n=2;MCHP.modsrc_id.id_11147.name='AFEC';MCHP.modsrc_id.id_11147.version='S';MCHP.modsrc_id.id_6417.n=1;MCHP.modsrc_id.id_6417.name='CHIPID';MCHP.modsrc_id.id_6417.version='ZK';MCHP.modsrc_id.id_11246.n=1;MCHP.modsrc_id.id_11246.name='DACC';MCHP.modsrc_id.id_11246.version='E';MCHP.modsrc_id.id_EBI.n=1;MCHP.modsrc_id.id_EBI.name='EBI';MCHP.modsrc_id.id_EBI.version='0';MCHP.modsrc_id.id_6450.n=1;MCHP.modsrc_id.id_6450.name='EFC';MCHP.modsrc_id.id_6450.version='Y';MCHP.modsrc_id.id_11046.n=1;MCHP.modsrc_id.id_11046.name='GMAC';MCHP.modsrc_id.id_11046.version='S';MCHP.modsrc_id.id_6378.n=1;MCHP.modsrc_id.id_6378.name='GPBR';MCHP.modsrc_id.id_6378.version='J';MCHP.modsrc_id.id_6449.n=1;MCHP.modsrc_id.id_6449.name='HSMCI';MCHP.modsrc_id.id_6449.version='R';MCHP.modsrc_id.id_11241.n=2;MCHP.modsrc_id.id_11241.name='I2SC';MCHP.modsrc_id.id_11241.version='N';MCHP.modsrc_id.id_11105.n=1;MCHP.modsrc_id.id_11105.name='ICM';MCHP.modsrc_id.id_11105.version='H';MCHP.modsrc_id.id_6350.n=1;MCHP.modsrc_id.id_6350.name='ISI';MCHP.modsrc_id.id_6350.version='K';MCHP.modsrc_id.id_11282.n=1;MCHP.modsrc_id.id_11282.name='MATRIX';MCHP.modsrc_id.id_11282.version='L';MCHP.modsrc_id.id_11273.n=2;MCHP.modsrc_id.id_11273.name='MCAN';MCHP.modsrc_id.id_11273.version='N';MCHP.modsrc_id.id_11004.n=5;MCHP.modsrc_id.id_11004.name='PIO';MCHP.modsrc_id.id_11004.version='V';MCHP.modsrc_id.id_44006.n=1;MCHP.modsrc_id.id_44006.name='PMC';MCHP.modsrc_id.id_44006.version='P';MCHP.modsrc_id.id_6343.n=2;MCHP.modsrc_id.id_6343.name='PWM';MCHP.modsrc_id.id_6343.version='Y';MCHP.modsrc_id.id_11171.n=1;MCHP.modsrc_id.id_11171.name='QSPI';MCHP.modsrc_id.id_11171.version='J';MCHP.modsrc_id.id_11009.n=1;MCHP.modsrc_id.id_11009.name='RSTC';MCHP.modsrc_id.id_11009.version='N';MCHP.modsrc_id.id_11110.n=1;MCHP.modsrc_id.id_11110.name='RSWDT';MCHP.modsrc_id.id_11110.version='G';MCHP.modsrc_id.id_6056.n=1;MCHP.modsrc_id.id_6056.name='RTC';MCHP.modsrc_id.id_6056.version='ZB';MCHP.modsrc_id.id_6081.n=1;MCHP.modsrc_id.id_6081.name='RTT';MCHP.modsrc_id.id_6081.version='M';MCHP.modsrc_id.id_6498.n=1;MCHP.modsrc_id.id_6498.name='SMC';MCHP.modsrc_id.id_6498.version='J';MCHP.modsrc_id.id_6088.n=2;MCHP.modsrc_id.id_6088.name='SPI';MCHP.modsrc_id.id_6088.version='ZM';MCHP.modsrc_id.id_6078.n=1;MCHP.modsrc_id.id_6078.name='SSC';MCHP.modsrc_id.id_6078.version='Q';MCHP.modsrc_id.id_6452.n=1;MCHP.modsrc_id.id_6452.name='SUPC';MCHP.modsrc_id.id_6452.version='ZE';MCHP.modsrc_id.id_6082.n=4;MCHP.modsrc_id.id_6082.name='TC';MCHP.modsrc_id.id_6082.version='ZL';MCHP.modsrc_id.id_6334.n=1;MCHP.modsrc_id.id_6334.name='TRNG';MCHP.modsrc_id.id_6334.version='G';MCHP.modsrc_id.id_11210.n=3;MCHP.modsrc_id.id_11210.name='TWIHS';MCHP.modsrc_id.id_11210.version='Z';MCHP.modsrc_id.id_6418.n=5;MCHP.modsrc_id.id_6418.name='UART';MCHP.modsrc_id.id_6418.version='R';MCHP.modsrc_id.id_6089.n=3;MCHP.modsrc_id.id_6089.name='USART';MCHP.modsrc_id.id_6089.version='ZW';MCHP.modsrc_id.id_11292.n=1;MCHP.modsrc_id.id_11292.name='USBHS';MCHP.modsrc_id.id_11292.version='G';MCHP.modsrc_id.id_11300.n=1;MCHP.modsrc_id.id_11300.name='UTMI';MCHP.modsrc_id.id_11300.version='A';MCHP.modsrc_id.id_6080.n=1;MCHP.modsrc_id.id_6080.name='WDT';MCHP.modsrc_id.id_6080.version='N';MCHP.modsrc_id.id_11161.n=1;MCHP.modsrc_id.id_11161.name='XDMAC';MCHP.modsrc_id.id_11161.version='K';MCHP.modsrc_id.id_1.n=1;MCHP.modsrc_id.id_1.name='LOCKBIT';MCHP.modsrc_id.id_1.version='1';MCHP.modsrc_id.id_SCnSCB.n=1;MCHP.modsrc_id.id_SCnSCB.name='SCnSCB';MCHP.modsrc_id.id_SCnSCB.version='0';MCHP.modsrc_id.id_SCB.n=1;MCHP.modsrc_id.id_SCB.name='SCB';MCHP.modsrc_id.id_SCB.version='0';MCHP.modsrc_id.id_SysTick.n=1;MCHP.modsrc_id.id_SysTick.name='SysTick';MCHP.modsrc_id.id_SysTick.version='0';MCHP.modsrc_id.id_NVIC.n=1;MCHP.modsrc_id.id_NVIC.name='NVIC';MCHP.modsrc_id.id_NVIC.version='0';MCHP.modsrc_id.id_MPU.n=1;MCHP.modsrc_id.id_MPU.name='MPU';MCHP.modsrc_id.id_MPU.version='0';MCHP.modsrc_id.id_FPU.n=1;MCHP.modsrc_id.id_FPU.name='FPU';MCHP.modsrc_id.id_FPU.version='0';MCHP.modsrc_id.id_ICE.n=1;MCHP.modsrc_id.id_ICE.name='ICE';MCHP.modsrc_id.id_ICE.version='0';MCHP.modsrc_id.id_TPIU.n=1;MCHP.modsrc_id.id_TPIU.name='TPIU';MCHP.modsrc_id.id_TPIU.version='0';MCHP.modsrc_Name.ACC.n=1;MCHP.modsrc_Name.ACC.id='6490';MCHP.modsrc_Name.ACC.version='J';MCHP.modsrc_Name.AES.n=1;MCHP.modsrc_Name.AES.id='6149';MCHP.modsrc_Name.AES.version='W';MCHP.modsrc_Name.AFEC.n=2;MCHP.modsrc_Name.AFEC.id='11147';MCHP.modsrc_Name.AFEC.version='S';MCHP.modsrc_Name.CHIPID.n=1;MCHP.modsrc_Name.CHIPID.id='6417';MCHP.modsrc_Name.CHIPID.version='ZK';MCHP.modsrc_Name.DACC.n=1;MCHP.modsrc_Name.DACC.id='11246';MCHP.modsrc_Name.DACC.version='E';MCHP.modsrc_Name.EBI.n=1;MCHP.modsrc_Name.EBI.id='EBI';MCHP.modsrc_Name.EBI.version='0';MCHP.modsrc_Name.EFC.n=1;MCHP.modsrc_Name.EFC.id='6450';MCHP.modsrc_Name.EFC.version='Y';MCHP.modsrc_Name.GMAC.n=1;MCHP.modsrc_Name.GMAC.id='11046';MCHP.modsrc_Name.GMAC.version='S';MCHP.modsrc_Name.GPBR.n=1;MCHP.modsrc_Name.GPBR.id='6378';MCHP.modsrc_Name.GPBR.version='J';MCHP.modsrc_Name.HSMCI.n=1;MCHP.modsrc_Name.HSMCI.id='6449';MCHP.modsrc_Name.HSMCI.version='R';MCHP.modsrc_Name.I2SC.n=2;MCHP.modsrc_Name.I2SC.id='11241';MCHP.modsrc_Name.I2SC.version='N';MCHP.modsrc_Name.ICM.n=1;MCHP.modsrc_Name.ICM.id='11105';MCHP.modsrc_Name.ICM.version='H';MCHP.modsrc_Name.ISI.n=1;MCHP.modsrc_Name.ISI.id='6350';MCHP.modsrc_Name.ISI.version='K';MCHP.modsrc_Name.MATRIX.n=1;MCHP.modsrc_Name.MATRIX.id='11282';MCHP.modsrc_Name.MATRIX.version='L';MCHP.modsrc_Name.MCAN.n=2;MCHP.modsrc_Name.MCAN.id='11273';MCHP.modsrc_Name.MCAN.version='N';MCHP.modsrc_Name.PIO.n=5;MCHP.modsrc_Name.PIO.id='11004';MCHP.modsrc_Name.PIO.version='V';MCHP.modsrc_Name.PMC.n=1;MCHP.modsrc_Name.PMC.id='44006';MCHP.modsrc_Name.PMC.version='P';MCHP.modsrc_Name.PWM.n=2;MCHP.modsrc_Name.PWM.id='6343';MCHP.modsrc_Name.PWM.version='Y';MCHP.modsrc_Name.QSPI.n=1;MCHP.modsrc_Name.QSPI.id='11171';MCHP.modsrc_Name.QSPI.version='J';MCHP.modsrc_Name.RSTC.n=1;MCHP.modsrc_Name.RSTC.id='11009';MCHP.modsrc_Name.RSTC.version='N';MCHP.modsrc_Name.RSWDT.n=1;MCHP.modsrc_Name.RSWDT.id='11110';MCHP.modsrc_Name.RSWDT.version='G';MCHP.modsrc_Name.RTC.n=1;MCHP.modsrc_Name.RTC.id='6056';MCHP.modsrc_Name.RTC.version='ZB';MCHP.modsrc_Name.RTT.n=1;MCHP.modsrc_Name.RTT.id='6081';MCHP.modsrc_Name.RTT.version='M';MCHP.modsrc_Name.SMC.n=1;MCHP.modsrc_Name.SMC.id='6498';MCHP.modsrc_Name.SMC.version='J';MCHP.modsrc_Name.SPI.n=2;MCHP.modsrc_Name.SPI.id='6088';MCHP.modsrc_Name.SPI.version='ZM';MCHP.modsrc_Name.SSC.n=1;MCHP.modsrc_Name.SSC.id='6078';MCHP.modsrc_Name.SSC.version='Q';MCHP.modsrc_Name.SUPC.n=1;MCHP.modsrc_Name.SUPC.id='6452';MCHP.modsrc_Name.SUPC.version='ZE';MCHP.modsrc_Name.TC.n=4;MCHP.modsrc_Name.TC.id='6082';MCHP.modsrc_Name.TC.version='ZL';MCHP.modsrc_Name.TRNG.n=1;MCHP.modsrc_Name.TRNG.id='6334';MCHP.modsrc_Name.TRNG.version='G';MCHP.modsrc_Name.TWIHS.n=3;MCHP.modsrc_Name.TWIHS.id='11210';MCHP.modsrc_Name.TWIHS.version='Z';MCHP.modsrc_Name.UART.n=5;MCHP.modsrc_Name.UART.id='6418';MCHP.modsrc_Name.UART.version='R';MCHP.modsrc_Name.USART.n=3;MCHP.modsrc_Name.USART.id='6089';MCHP.modsrc_Name.USART.version='ZW';MCHP.modsrc_Name.USBHS.n=1;MCHP.modsrc_Name.USBHS.id='11292';MCHP.modsrc_Name.USBHS.version='G';MCHP.modsrc_Name.UTMI.n=1;MCHP.modsrc_Name.UTMI.id='11300';MCHP.modsrc_Name.UTMI.version='A';MCHP.modsrc_Name.WDT.n=1;MCHP.modsrc_Name.WDT.id='6080';MCHP.modsrc_Name.WDT.version='N';MCHP.modsrc_Name.XDMAC.n=1;MCHP.modsrc_Name.XDMAC.id='11161';MCHP.modsrc_Name.XDMAC.version='K';MCHP.modsrc_Name.FUSES.n=1;MCHP.modsrc_Name.FUSES.id='1';MCHP.modsrc_Name.FUSES.version='1';MCHP.modsrc_Name.LOCKBIT.n=1;MCHP.modsrc_Name.LOCKBIT.id='1';MCHP.modsrc_Name.LOCKBIT.version='1';MCHP.modsrc_Name.SCnSCB.n=1;MCHP.modsrc_Name.SCnSCB.id='SCnSCB';MCHP.modsrc_Name.SCnSCB.version='0';MCHP.modsrc_Name.SCB.n=1;MCHP.modsrc_Name.SCB.id='SCB';MCHP.modsrc_Name.SCB.version='0';MCHP.modsrc_Name.SysTick.n=1;MCHP.modsrc_Name.SysTick.id='SysTick';MCHP.modsrc_Name.SysTick.version='0';MCHP.modsrc_Name.NVIC.n=1;MCHP.modsrc_Name.NVIC.id='NVIC';MCHP.modsrc_Name.NVIC.version='0';MCHP.modsrc_Name.MPU.n=1;MCHP.modsrc_Name.MPU.id='MPU';MCHP.modsrc_Name.MPU.version='0';MCHP.modsrc_Name.FPU.n=1;MCHP.modsrc_Name.FPU.id='FPU';MCHP.modsrc_Name.FPU.version='0';MCHP.modsrc_Name.ICE.n=1;MCHP.modsrc_Name.ICE.id='ICE';MCHP.modsrc_Name.ICE.version='0';MCHP.modsrc_Name.TPIU.n=1;MCHP.modsrc_Name.TPIU.id='TPIU';MCHP.modsrc_Name.TPIU.version='0';MCHP.PortBase=32;MCHP.PortPrefixe='P';MCHP.PowerSave=0;MCHP.fcy.MIPS=3e+08;MCHP.fcy.MCK=1.5e+08;MCHP.fcy.Timers=1.5e+08;MCHP.fcy.SUPC=1.5e+08;MCHP.fcy.RSTC=1.5e+08;MCHP.fcy.RTC=1.5e+08;MCHP.fcy.RTT=1.5e+08;MCHP.fcy.WDT=1.5e+08;MCHP.fcy.PMC=1.5e+08;MCHP.fcy.EFC=1.5e+08;MCHP.fcy.UART0=1.5e+08;MCHP.fcy.UART1=1.5e+08;MCHP.fcy.PIOA=1.5e+08;MCHP.fcy.PIOB=1.5e+08;MCHP.fcy.PIOC=1.5e+08;MCHP.fcy.USART0=1.5e+08;MCHP.fcy.USART1=1.5e+08;MCHP.fcy.USART2=1.5e+08;MCHP.fcy.PIOD=1.5e+08;MCHP.fcy.PIOE=1.5e+08;MCHP.fcy.HSMCI=1.5e+08;MCHP.fcy.TWIHS0=1.5e+08;MCHP.fcy.TWIHS1=1.5e+08;MCHP.fcy.SPI0=1.5e+08;MCHP.fcy.SSC=1.5e+08;MCHP.fcy.TC0=1.5e+08;MCHP.fcy.TC1=1.5e+08;MCHP.fcy.AFEC0=1.5e+08;MCHP.fcy.DACC=1.5e+08;MCHP.fcy.PWM0=1.5e+08;MCHP.fcy.ICM=1.5e+08;MCHP.fcy.ACC=1.5e+08;MCHP.fcy.USBHS=1.5e+08;MCHP.fcy.MCAN0=1.5e+08;MCHP.fcy.MCAN1=1.5e+08;MCHP.fcy.GMAC=1.5e+08;MCHP.fcy.AFEC1=1.5e+08;MCHP.fcy.TWIHS2=1.5e+08;MCHP.fcy.SPI1=1.5e+08;MCHP.fcy.QSPI=1.5e+08;MCHP.fcy.UART2=1.5e+08;MCHP.fcy.UART3=1.5e+08;MCHP.fcy.UART4=1.5e+08;MCHP.fcy.TC2=1.5e+08;MCHP.fcy.TC3=1.5e+08;MCHP.fcy.AES=1.5e+08;MCHP.fcy.TRNG=1.5e+08;MCHP.fcy.XDMAC=1.5e+08;MCHP.fcy.ISI=1.5e+08;MCHP.fcy.PWM1=1.5e+08;MCHP.fcy.FPU=1.5e+08;MCHP.fcy.RSWDT=1.5e+08;MCHP.fcy.SCB=1.5e+08;MCHP.fcy.I2SC0=1.5e+08;MCHP.fcy.I2SC1=1.5e+08;MCHP.fcy.EBI=1.5e+08;MCHP.fcy.ICE=1.5e+08;MCHP.fcy.TPIU=1.5e+08;MCHP.fcy.FUSES=1.5e+08;MCHP.NTIMERS=12;MCHP.SCCP.nSCCP=0;MCHP.SYS_TICK_TS_Load=299999;MCHP.TimeStepFactor=1;MCHP.INT_PRIORITY_DMA='7';  MCHP_CRC=37746645  BTMODE=Device is in Single Boot (legacy) mode  RES1=Not used  PLLSS=Not used  RES2=Not used  ALTCMPI=Not used  BOREN1=Not used  ALTRB6=Not used  RETCFG=Not used  DFMCY=Not used  BSS2=No Boot Segment  BSEN=No Boot Segment  CWRP=Configuration Segment may be written  CSS=No Protection (other than CWRP)  AIVTDIS=Disable Alternate Vector Table  BSLIM=Not used  WDTEN=Disable  BTSWP=BOOTSWP instruction is disabled  DBCC=No Cross Connection between DAC outputs  CTXT1=Not Assigned  CTXT2=Not Assigned  SEQNUM=Not used  nSEQNUM=Not used  BOREN0=Enabled  DMTIVT=Not used  DMTCNT=2^31 (2147483648)  DMTEN=Dead Man Timer is Disabled and can be enabled by software  ON=Not used  USERID=Not used  RESERVED1=Not used  PGL1WAY=Allow only one reconfiguration  FPLLRNG=34-68 MHz Input  FPLLICLK=FRC is input to the System PLL  FPLLMULT=PLL Multiply by 128  UPLLFSEL=USB PLL input is 24 MHz  DMTINTV=Window/Interval value is 127/128 counter value  WDTSPGM=WDT stops during Flash programming  FDMTEN=Deadman Timer is disabled  TRCEN=Trace features in the CPU are enabled  BOOTISA=Boot code and Exception code is MIPS32  FECCCON=ECC and Dynamic ECC are disabled (ECCCON bits are writable)  EXTDDRSIZE=Not used  FSLEEP=Flash is powered down when the device is in Sleep mode  DBGPER=Allow CPU access to all permission regions  EJTAGBEN=Normal EJTAG functionality  TSEQ=Not used  CSEQ=Not used  RWDTPS=1:1048576  RCLKSEL=Always use LPRC  SWDTPS=1:1048576  DMTIVTL=Not used  DMTIVTH=Not used  DMTCNTL=Not used  DMTCNTH=Not used  DMTDIS=Dead Man Timer is Disabled and can be enabled by software  SMBEN=SMBus input threshold is enabled  SPI2PIN=SPI2 uses I/O remap (PPS) pins  CTXT3=Not Assigned  CTXT4=Not Assigned  MBXM0=Mailbox register configured for Main data read (Secondary to Main data transfer)  MBXM1=Mailbox register configured for Main data read (Secondary to Main data transfer)  MBXM2=Mailbox register configured for Main data read (Secondary to Main data transfer)  MBXM3=Mailbox register configured for Main data read (Secondary to Main data transfer)  MBXM4=Mailbox register configured for Main data read (Secondary to Main data transfer)  MBXM5=Mailbox register configured for Main data read (Secondary to Main data transfer)  MBXM6=Mailbox register configured for Main data read (Secondary to Main data transfer)  MBXM7=Mailbox register configured for Main data read (Secondary to Main data transfer)  MBXM8=Mailbox register configured for Main data read (Secondary to Main data transfer)  MBXM9=Mailbox register configured for Main data read (Secondary to Main data transfer)  MBXM10=Mailbox register configured for Main data read (Secondary to Main data transfer)  MBXM11=Mailbox register configured for Main data read (Secondary to Main data transfer)  MBXM12=Mailbox register configured for Main data read (Secondary to Main data transfer)  MBXM13=Mailbox register configured for Main data read (Secondary to Main data transfer)  MBXM14=Mailbox register configured for Main data read (Secondary to Main data transfer)  MBXM15=Mailbox register configured for Main data read (Secondary to Main data transfer)  MBXHSA=MSIxMBXD15 assigned to mailbox handshake protocol block A  MBXHSB=MSIxMBXD15 assigned to mailbox handshake protocol block B  MBXHSC=MSIxMBXD15 assigned to mailbox handshake protocol block C  MBXHSD=MSIxMBXD15 assigned to mailbox handshake protocol block D  MBXHSE=MSIxMBXD15 assigned to mailbox handshake protocol block E  MBXHSF=MSIxMBXD15 assigned to mailbox handshake protocol block F  MBXHSG=MSIxMBXD15 assigned to mailbox handshake protocol block G  MBXHSH=MSIxMBXD15 assigned to mailbox handshake protocol block H  HSAEN=Mailbox data flow control handshake protocol block disabled  HSBEN=Mailbox data flow control handshake protocol block disabled  HSCEN=Mailbox data flow control handshake protocol block disabled  HSDEN=Mailbox data flow control handshake protocol block disabled  HSEEN=Mailbox data flow control handshake protocol block disabled  HSFEN=Mailbox data flow control handshake protocol block disabled  HSGEN=Mailbox data flow control handshake protocol block disabled  HSHEN=Mailbox data flow control handshake protocol block disabled  CPRA0=Main core owns pin  CPRA1=Main core owns pin  CPRA2=Main core owns pin  CPRA3=Main core owns pin  CPRA4=Main core owns pin  CPRB0=Main core owns pin  CPRB1=Main core owns pin  CPRB2=Main core owns pin  CPRB3=Main core owns pin  CPRB4=Main core owns pin  CPRB5=Main core owns pin  CPRB6=Main core owns pin  CPRB7=Main core owns pin  CPRB8=Main core owns pin  CPRB9=Main core owns pin  CPRB10=Main core owns pin  CPRB11=Main core owns pin  CPRB12=Main core owns pin  CPRB13=Main core owns pin  CPRB14=Main core owns pin  CPRB15=Main core owns pin  CPRC0=Main core owns pin  CPRC1=Main core owns pin  CPRC2=Main core owns pin  CPRC3=Main core owns pin  CPRC4=Main core owns pin  CPRC5=Main core owns pin  CPRC6=Main core owns pin  CPRC7=Main core owns pin  CPRC8=Main core owns pin  CPRC9=Main core owns pin  CPRC10=Main core owns pin  CPRC11=Main core owns pin  CPRC12=Main core owns pin  CPRC13=Main core owns pin  CPRC14=Main core owns pin  CPRC15=Main core owns pin  CPRD0=Main core owns pin  CPRD1=Main core owns pin  CPRD2=Main core owns pin  CPRD3=Main core owns pin  CPRD4=Main core owns pin  CPRD5=Main core owns pin  CPRD6=Main core owns pin  CPRD7=Main core owns pin  CPRD8=Main core owns pin  CPRD9=Main core owns pin  CPRD10=Main core owns pin  CPRD11=Main core owns pin  CPRD12=Main core owns pin  CPRD13=Main core owns pin  CPRD14=Main core owns pin  CPRD15=Main core owns pin  CPRE0=Main core owns pin  CPRE1=Main core owns pin  CPRE2=Main core owns pin  CPRE3=Main core owns pin  CPRE4=Main core owns pin  CPRE5=Main core owns pin  CPRE6=Main core owns pin  CPRE7=Main core owns pin  CPRE8=Main core owns pin  CPRE9=Main core owns pin  CPRE10=Main core owns pin  CPRE11=Main core owns pin  CPRE12=Main core owns pin  CPRE13=Main core owns pin  CPRE14=Main core owns pin  CPRE15=Main core owns pin  S1FNOSC=Internal Fast RC (FRC) Oscillator with postscaler  S1IESO=Start up with FRC; then switch  S1OSCIOFNC=OSC2 is clock output  S1FCKSM=Both Clock switching and Fail-safe Clock Monitor are disabled  S1PLLKEN=S1PLLKEN_ON  S1RWDTPS=1:1048576  S1RCLKSEL=Always use LPRC  S1WINDIS=Watchdog Timer operates in Non-Window mode  S1WDTWIN=WDT Window is 25% of WDT period  S1SWDTPS=1:1048576  S1FWDTEN=use WDTCON.ON bit  S1ICS=Communicate on PGC1 and PGD1  S1DEBUG=Not used  S1ISOLAT=The Secondary can operate (in debug mode) even if the SLVEN bit in the MSI is zero  S1NOBTSWP=BOOTSWP instruction is disabled  S1ALTI2C1=I2C1 mapped to SDA1/SCL1 pins  S1SPI1PIN=Secondary SPI1 uses I/O remap (PPS) pins  S1SSRE=Secondary generated resets will reset the Secondary Enable Bit in the MSI module  S1MSRE=The Main software oriented RESET events (RESET Op-Code; Watchdog timeout; TRAP reset; illegalInstruction) will also cause the Secondary subsystem to reset  S1CTXT1=Not Assigned  S1CTXT2=Not Assigned  S1CTXT3=Not Assigned  S1CTXT4=Not Assigned  BORLVL=BOR trip point is 2.96 V  BSSO=Normal startup operation after reset; execute instruction at 0x000000  MCA=Flash read accesses are 2 cycle to support maximum processor frequency of operation  MAXTEMP=20 ns flash access  CFGAN14=Device pin is input to AN14  CFGAN15=Device pin is input to AN15  S1IOL1WAY=Allow only one reconfiguration  S1BSSO=Normal startup operation after reset; execute instruction at 0x000000  S1BACKBUG=Not used  BISTDIS=mBIST on reset feature disabled  NOBTSWP=BOOTSWP instruction is disabled  S1BISTDIS=Secondary BIST on reset feature disabled  S1DMTIVTL=Not used  S1DMTIVTH=Not used  S1DMTCNTL=Not used  S1DMTCNTH=Not used  S1DMTDIS=Secondary Dead Man Timer is Disabled and can be enabled by software  BSEQ=Not used  IBSEQ=Not used  SMB3EN=SMBus 3.0 input levels  FUSBIDIO2=USBID pin is controlled by the USB2 module  FVBUSIO2=VBUSON pin is controlled by the USB2 module  FUSBIDIO1=USBID pin is controlled by the USB1 module  FVBUSIO1=VBUSON pin is controlled by the USB1 module  VBATBOREN=Enable ZPBOR during VBAT Mode  FDSEN=Enable DSEN bit in DSCON  BORSEL=BOR trip voltage 2.1v (Non-OPAMP deviced operation)  POSCFGAIN=Gain is G3  POSCAGCDLY=Settling time = 25ms x AGCRNG  POSCAGCRNG=Range 1x  POSCAGC=Automatic Gain Control for Oscillator  FDBGWP=Not used
      settings: SourceProductName=MPLAB Device Blocks for Simulink
  Port Info : MCHP_Blockset/System Info/Port Info  MCHP_MASTERLINK=mcb_microchip_pmsm_parameter_est_SAME70_23b_lib/Microcontroller/Configurations/Microchip Master
      settings: SourceProductName=MPLAB Device Blocks for Simulink
  UART Configuration : MCHP_Blockset/BUS UART/UART Configuration  UART_REF=UART 0  BAUD_Choice=Dynamic Options  BAUD_Choice_TXT="1200000         [-2.34%]"  BAUD_Choice_IR=Dynamic Options  BAUD_Choice_IR_TXT=[]  BAUD_Custom=115200  INT_PRIORITY=3  ALT_IO=on  PIN_RX=Dynamic Options  PIN_RX_TXT=PA9 / Pin[75]  PIN_TX=Dynamic Options  PIN_TX_TXT=PA10 / Pin[66]  MCHP_PORT={UART 0 Rx}{URXD0}3:0:P9;{UART 0 Tx}{UTXD0}3:1:P10;  MCHP_MASTERLINK=mcb_microchip_pmsm_parameter_est_SAME70_23b_lib/Microcontroller/Configurations/Microchip Master  MCHP_COM_ExtPil=off  TX_IMPLEMENTATION=DMA Ping-Pong Mode  TX_IMPLEMENTATION_default=Circular Buffer  TX_INT_PRIORITY=5  TX_INT_WHEN=is empty  TX_INT_WHEN_default=is empty & last char is sent  TX_CIRCULAR_SIZE=128  TX_DMA_CHANNEL=0  TX_DMA_SIZE=120*4+2  TX_TASK_PROTECTION=Delay tasks (default)  TX_INTERRUPT_PROTECTION=Do not send on conflict (default)  TX_INTERRUPT_PROTECTION_default=Do not send on conflict (default)  RX_IMPLEMENTATION=Circular Buffer  RX_IMPLEMENTATION_default=Circular Buffer  RX_INT_PRIORITY=5  RX_INT_WHEN=is full (contains 4 data characters)  RX_CIRCULAR_SIZE=32  RX_DMA_CHANNEL=0  RX_DMA_SIZE=0  DuplexMode=Full duplex (default)  PIN_RX_Inv=off  PIN_TX_Inv=off  PIN_RXTX_Inv=off  ParityBit=No parity (default)  StopBit=1 stop bit (default)  IRDA=off  IdleTime_choice=Dynamic Options  IdleTime_choice_TXT=0  IdleTime_custom=2/50  FlowControl=None  PIN_CTS=Dynamic Options  PIN_CTS_TXT=PD19 / Pin[67]  PIN_RTS=Dynamic Options  PIN_RTS_TXT=PD18 / Pin[69]  PIN_DSR=Dynamic Options  PIN_DSR_TXT=Dynamic Options  PIN_DTR=Dynamic Options  PIN_DTR_TXT=Dynamic Options  InitSequence_chkbox=off  BAUD_Choice_InitSeq=Dynamic Options  BAUD_Choice_InitSeq_TXT="110         [+30.05%]"  BAUD_Choice_IR_InitSeq=Dynamic Options  BAUD_Choice_IR_InitSeq_TXT=0  BAUD_Custom_InitSeq=0  InitSequence='Hello World'
      settings: SourceProductName=MPLAB Device Blocks for Simulink
